simulink model "model"  (R2014a)
(part 5 of 5)

  T_166670638__/LConn2 -- _CN_166670638_220000_CN_166785368_220000/LConn2
  _CN_166670638_220000_CN_166785368_220000/LConn3 -- T_166670638__/LConn3 -- bus177/LConn1
  _CN_166670638_220000_CN_166785368_220000/RConn1 -- T_166785368__/LConn1 -- _CN_287217193_220000_CN_166785368_220000/LConn1
  _CN_166670638_220000_CN_166785368_220000/RConn2 -- T_166785368__/LConn2 -- _CN_287217193_220000_CN_166785368_220000/LConn2
  _CN_166670638_220000_CN_166785368_220000/RConn3 -- T_166785368__/LConn3 -- _CN_287217193_220000_CN_166785368_220000/LConn3 -- bus178/LConn1
  T_105834287__/LConn1 -- _CN_105834287_220000_CN_121056862_220000/RConn1
  T_105834287__/LConn2 -- _CN_105834287_220000_CN_121056862_220000/RConn2
  _CN_105834287_220000_CN_121056862_220000/RConn3 -- T_105834287__/LConn3 -- bus179/LConn1
  T_162167601__/LConn1 -- _CN_162167601_220000_CN_162167607_220000/LConn1
  T_162167601__/LConn2 -- _CN_162167601_220000_CN_162167607_220000/LConn2
  _CN_162167601_220000_CN_162167607_220000/LConn3 -- T_162167601__/LConn3 -- bus180/LConn1
  _CN_162167601_220000_CN_162167607_220000/RConn1 -- T_162167607__/LConn1 -- _CN_162167607_220000_CN_286930814_220000/LConn1 -- _CN_162167607_220000_CN_162378099_220000/RConn1
  _CN_162167601_220000_CN_162167607_220000/RConn2 -- T_162167607__/LConn2 -- _CN_162167607_220000_CN_286930814_220000/LConn2 -- _CN_162167607_220000_CN_162378099_220000/RConn2
  _CN_162167601_220000_CN_162167607_220000/RConn3 -- T_162167607__/LConn3 -- _CN_162167607_220000_CN_286930814_220000/LConn3 -- _CN_162167607_220000_CN_162378099_220000/RConn3 -- bus181/LConn1
  T_166785367__/LConn1 -- _CN_166670643_220000_CN_166785367_220000/RConn1
  T_166785367__/LConn2 -- _CN_166670643_220000_CN_166785367_220000/RConn2
  _CN_166670643_220000_CN_166785367_220000/RConn3 -- T_166785367__/LConn3 -- bus182/LConn1
  _CN_167981876_220000_CN_148003696_220000/LConn1 -- T_167981876_500000_/RConn1 -- L_167981876/LConn1
  _CN_167981876_220000_CN_148003696_220000/LConn2 -- T_167981876_500000_/RConn2 -- L_167981876/LConn2
  _CN_167981876_220000_CN_148003696_220000/LConn3 -- T_167981876_500000_/RConn3 -- L_167981876/LConn3 -- bus183/LConn1
  T_148003696__/LConn1 -- _CN_167981876_220000_CN_148003696_220000/RConn1
  T_148003696__/LConn2 -- _CN_167981876_220000_CN_148003696_220000/RConn2
  _CN_167981876_220000_CN_148003696_220000/RConn3 -- T_148003696__/LConn3 -- bus184/LConn1
  _CN_162167607_220000_CN_286930814_220000/RConn1 -- T_286930814__/LConn1 -- _CN_286930852_220000_CN_286930814_220000/RConn1
  _CN_162167607_220000_CN_286930814_220000/RConn2 -- T_286930814__/LConn2 -- _CN_286930852_220000_CN_286930814_220000/RConn2
  _CN_162167607_220000_CN_286930814_220000/RConn3 -- T_286930814__/LConn3 -- _CN_286930852_220000_CN_286930814_220000/RConn3 -- bus185/LConn1
  T_132430141__/LConn1 -- _CN_132430137_220000_CN_132430141_220000/RConn1
  T_132430141__/LConn2 -- _CN_132430137_220000_CN_132430141_220000/RConn2
  _CN_132430137_220000_CN_132430141_220000/RConn3 -- T_132430141__/LConn3 -- bus186/LConn1
  _CN_287217193_220000_CN_166670647_220000/LConn1 -- T_287217193__/LConn1 -- _CN_287217193_220000_CN_166785368_220000/RConn1 -- _CN_287217193_220000_CN_287217195_220000/LConn1
  _CN_287217193_220000_CN_166670647_220000/LConn2 -- T_287217193__/LConn2 -- _CN_287217193_220000_CN_166785368_220000/RConn2 -- _CN_287217193_220000_CN_287217195_220000/LConn2
  _CN_287217193_220000_CN_166670647_220000/LConn3 -- T_287217193__/LConn3 -- _CN_287217193_220000_CN_166785368_220000/RConn3 -- _CN_287217193_220000_CN_287217195_220000/LConn3 -- bus187/LConn1
  _CN_287217193_220000_CN_166670647_220000/RConn1 -- G_166670647_/RConn1 -- _CN_166670597_500000_CN_166670647_220000/LConn1
  _CN_287217193_220000_CN_166670647_220000/RConn2 -- G_166670647_/RConn2 -- _CN_166670597_500000_CN_166670647_220000/LConn2
  _CN_287217193_220000_CN_166670647_220000/RConn3 -- G_166670647_/RConn3 -- _CN_166670597_500000_CN_166670647_220000/LConn3 -- bus188/LConn1
  T_287217195__/LConn1 -- _CN_287217193_220000_CN_287217195_220000/RConn1
  T_287217195__/LConn2 -- _CN_287217193_220000_CN_287217195_220000/RConn2
  _CN_287217193_220000_CN_287217195_220000/RConn3 -- T_287217195__/LConn3 -- bus189/LConn1
  T_107081025_220000_/LConn1 -- _CN_107081025_220000_CN_107081068_220000/LConn1
  T_107081025_220000_/LConn2 -- _CN_107081025_220000_CN_107081068_220000/LConn2
  _CN_107081025_220000_CN_107081068_220000/LConn3 -- T_107081025_220000_/LConn3 -- bus190/LConn1
  _CN_107081025_220000_CN_107081068_220000/RConn1 -- G_107081068_吴泾热电站/RConn1 -- _CN_107081079_220000_CN_107081068_220000/LConn1
  _CN_107081025_220000_CN_107081068_220000/RConn2 -- G_107081068_吴泾热电站/RConn2 -- _CN_107081079_220000_CN_107081068_220000/LConn2
  _CN_107081025_220000_CN_107081068_220000/RConn3 -- G_107081068_吴泾热电站/RConn3 -- _CN_107081079_220000_CN_107081068_220000/LConn3 -- bus191/LConn1
  _CN_107025734_220000_CN_107025738_220000/LConn1 -- T_107025734__/LConn1 -- _CN_107025734_220000_CN_95805677_220000/RConn1
  _CN_107025734_220000_CN_107025738_220000/LConn2 -- T_107025734__/LConn2 -- _CN_107025734_220000_CN_95805677_220000/RConn2
  _CN_107025734_220000_CN_107025738_220000/LConn3 -- T_107025734__/LConn3 -- _CN_107025734_220000_CN_95805677_220000/RConn3 -- bus192/LConn1
  T_107025738__/LConn1 -- _CN_107025734_220000_CN_107025738_220000/RConn1
  T_107025738__/LConn2 -- _CN_107025734_220000_CN_107025738_220000/RConn2
  _CN_107025734_220000_CN_107025738_220000/RConn3 -- T_107025738__/LConn3 -- bus193/LConn1
  T_148630855__/LConn1 -- _CN_148630855_220000_CN_148630906_220000/LConn1
  T_148630855__/LConn2 -- _CN_148630855_220000_CN_148630906_220000/LConn2
  _CN_148630855_220000_CN_148630906_220000/LConn3 -- T_148630855__/LConn3 -- bus194/LConn1
  T_148630906__/LConn1 -- _CN_148630855_220000_CN_148630906_220000/RConn1
  T_148630906__/LConn2 -- _CN_148630855_220000_CN_148630906_220000/RConn2
  _CN_148630855_220000_CN_148630906_220000/RConn3 -- T_148630906__/LConn3 -- bus195/LConn1
  _CN_163357515_220000_CN_165791616_220000/LConn1 -- T_163357515__/RConn1 -- L_163357515/LConn1
  _CN_163357515_220000_CN_165791616_220000/LConn2 -- T_163357515__/RConn2 -- L_163357515/LConn2
  _CN_163357515_220000_CN_165791616_220000/LConn3 -- T_163357515__/RConn3 -- L_163357515/LConn3 -- bus196/LConn1
  T_165791616__/LConn1 -- _CN_163357515_220000_CN_165791616_220000/RConn1
  T_165791616__/LConn2 -- _CN_163357515_220000_CN_165791616_220000/RConn2
  _CN_163357515_220000_CN_165791616_220000/RConn3 -- T_165791616__/LConn3 -- bus197/LConn1
  _CN_355642647_220000_CN_313585533_220000/RConn1 -- T_313585533_220000_/LConn1 -- _CN_313585532_220000_CN_313585533_220000/RConn1
  _CN_355642647_220000_CN_313585533_220000/RConn2 -- T_313585533_220000_/LConn2 -- _CN_313585532_220000_CN_313585533_220000/RConn2
  _CN_355642647_220000_CN_313585533_220000/RConn3 -- T_313585533_220000_/LConn3 -- _CN_313585532_220000_CN_313585533_220000/RConn3 -- bus198/LConn1
  T_439464430__/LConn1 -- _CN_355642647_220000_CN_439464430_220000/RConn1
  T_439464430__/LConn2 -- _CN_355642647_220000_CN_439464430_220000/RConn2
  _CN_355642647_220000_CN_439464430_220000/RConn3 -- T_439464430__/LConn3 -- bus199/LConn1
  T_276589719__/LConn1 -- _CN_312789337_220000_CN_276589719_220000/RConn1
  T_276589719__/LConn2 -- _CN_312789337_220000_CN_276589719_220000/RConn2
  _CN_312789337_220000_CN_276589719_220000/RConn3 -- T_276589719__/LConn3 -- bus200/LConn1
  T_107025757_220000_/LConn1 -- _CN_107025757_220000_CN_95805677_220000/RConn1
  T_107025757_220000_/LConn2 -- _CN_107025757_220000_CN_95805677_220000/RConn2
  _CN_107025757_220000_CN_95805677_220000/RConn3 -- T_107025757_220000_/LConn3 -- bus201/LConn1
  T_137158504_220000_/LConn1 -- _CN_137158504_220000_CN_373557043_220000/LConn1
  T_137158504_220000_/LConn2 -- _CN_137158504_220000_CN_373557043_220000/LConn2
  _CN_137158504_220000_CN_373557043_220000/LConn3 -- T_137158504_220000_/LConn3 -- bus202/LConn1
  G_373557043_/RConn1 -- _CN_137158504_220000_CN_373557043_220000/RConn1
  G_373557043_/RConn2 -- _CN_137158504_220000_CN_373557043_220000/RConn2
  _CN_137158504_220000_CN_373557043_220000/RConn3 -- G_373557043_/RConn3 -- bus203/LConn1
  T_286930806__/LConn1 -- _CN_286930806_220000_CN_286930848_220000/LConn1
  T_286930806__/LConn2 -- _CN_286930806_220000_CN_286930848_220000/LConn2
  _CN_286930806_220000_CN_286930848_220000/LConn3 -- T_286930806__/LConn3 -- bus204/LConn1
  _CN_286930806_220000_CN_286930848_220000/RConn1 -- T_286930848__/LConn1 -- _CN_286930848_220000_CN_286930851_220000/LConn1
  _CN_286930806_220000_CN_286930848_220000/RConn2 -- T_286930848__/LConn2 -- _CN_286930848_220000_CN_286930851_220000/LConn2
  _CN_286930806_220000_CN_286930848_220000/RConn3 -- T_286930848__/LConn3 -- _CN_286930848_220000_CN_286930851_220000/LConn3 -- bus205/LConn1
  _CN_107081079_220000_CN_107081068_220000/RConn1 -- T_107081079_220000_/LConn1 -- _CN_107081079_220000_CN_95805677_220000/RConn1
  _CN_107081079_220000_CN_107081068_220000/RConn2 -- T_107081079_220000_/LConn2 -- _CN_107081079_220000_CN_95805677_220000/RConn2
  _CN_107081079_220000_CN_107081068_220000/RConn3 -- T_107081079_220000_/LConn3 -- _CN_107081079_220000_CN_95805677_220000/RConn3 -- bus206/LConn1
  T_201195907_220000_/LConn1 -- _CN_201195906_220000_CN_201195907_220000/RConn1
  T_201195907_220000_/LConn2 -- _CN_201195906_220000_CN_201195907_220000/RConn2
  _CN_201195906_220000_CN_201195907_220000/RConn3 -- T_201195907_220000_/LConn3 -- bus207/LConn1
  _CN_283658124_220000_CN_284090317_220000/LConn1 -- T_283658124__/RConn1 -- L_283658124/LConn1
  _CN_283658124_220000_CN_284090317_220000/LConn2 -- T_283658124__/RConn2 -- L_283658124/LConn2
  _CN_283658124_220000_CN_284090317_220000/LConn3 -- T_283658124__/RConn3 -- L_283658124/LConn3 -- bus208/LConn1
  _CN_283658124_220000_CN_284090317_220000/RConn1 -- T_284090317__/LConn1 -- _CN_284090317_220000_CN_284090323_220000/LConn1
  _CN_283658124_220000_CN_284090317_220000/RConn2 -- T_284090317__/LConn2 -- _CN_284090317_220000_CN_284090323_220000/LConn2
  _CN_283658124_220000_CN_284090317_220000/RConn3 -- T_284090317__/LConn3 -- _CN_284090317_220000_CN_284090323_220000/LConn3 -- bus209/LConn1
  _CN_128731545_220000_CN_132311997_220000/LConn1 -- T_128731545_220000_/LConn1 -- _CN_128731545_220000_CN_132312010_220000/RConn1 -- _CN_128731545_220000_CN_128731546_220000/RConn1
  _CN_128731545_220000_CN_132311997_220000/LConn2 -- T_128731545_220000_/LConn2 -- _CN_128731545_220000_CN_132312010_220000/RConn2 -- _CN_128731545_220000_CN_128731546_220000/RConn2
  _CN_128731545_220000_CN_132311997_220000/LConn3 -- T_128731545_220000_/LConn3 -- _CN_128731545_220000_CN_132312010_220000/RConn3 -- bus210/LConn1 -- _CN_128731545_220000_CN_128731546_220000/RConn3
  _CN_128731545_220000_CN_132311997_220000/RConn1 -- T_132311997_220000_/LConn1 -- _CN_132311997_220000_CN_132312010_220000/RConn1
  _CN_128731545_220000_CN_132311997_220000/RConn2 -- T_132311997_220000_/LConn2 -- _CN_132311997_220000_CN_132312010_220000/RConn2
  _CN_128731545_220000_CN_132311997_220000/RConn3 -- T_132311997_220000_/LConn3 -- _CN_132311997_220000_CN_132312010_220000/RConn3 -- bus211/LConn1
  T_286930851__/LConn1 -- _CN_286930848_220000_CN_286930851_220000/RConn1
  T_286930851__/LConn2 -- _CN_286930848_220000_CN_286930851_220000/RConn2
  _CN_286930848_220000_CN_286930851_220000/RConn3 -- T_286930851__/LConn3 -- bus212/LConn1
  T_223960988__/LConn1 -- _CN_223960988_220000_CN_337055172_220000/LConn1
  T_223960988__/LConn2 -- _CN_223960988_220000_CN_337055172_220000/LConn2
  _CN_223960988_220000_CN_337055172_220000/LConn3 -- T_223960988__/LConn3 -- bus213/LConn1
  T_337055172_500000_/LConn1 -- _CN_223960988_220000_CN_337055172_220000/RConn1
  T_337055172_500000_/LConn2 -- _CN_223960988_220000_CN_337055172_220000/RConn2
  _CN_223960988_220000_CN_337055172_220000/RConn3 -- T_337055172_500000_/LConn3 -- bus214/LConn1
  T_314318262_220000_/LConn1 -- _CN_314318262_220000_CN_314288467_220000/RConn1
  T_314318262_220000_/LConn2 -- _CN_314318262_220000_CN_314288467_220000/RConn2
  _CN_314318262_220000_CN_314288467_220000/RConn3 -- T_314318262_220000_/LConn3 -- bus215/LConn1
  T_284090323__/LConn1 -- _CN_284090317_220000_CN_284090323_220000/RConn1
  T_284090323__/LConn2 -- _CN_284090317_220000_CN_284090323_220000/RConn2
  _CN_284090317_220000_CN_284090323_220000/RConn3 -- T_284090323__/LConn3 -- bus216/LConn1
  T_163985922__/LConn1 -- _CN_163985922_500000_CN_127871762_500000/LConn1
  T_163985922__/LConn2 -- _CN_163985922_500000_CN_127871762_500000/LConn2
  _CN_163985922_500000_CN_127871762_500000/LConn3 -- T_163985922__/LConn3 -- bus217/LConn1
  T_127871762_500000_/LConn1 -- _CN_163985922_500000_CN_127871762_500000/RConn1
  T_127871762_500000_/LConn2 -- _CN_163985922_500000_CN_127871762_500000/RConn2
  _CN_163985922_500000_CN_127871762_500000/RConn3 -- T_127871762_500000_/LConn3 -- bus218/LConn1
  _CN_287200264_500000_CN_312588760_500000/LConn1 -- T_287200264__/LConn1 -- _CN_287200264_500000_CN_28939657_500000/LConn1 -- _CN_287200264_500000_CN_287132220_500000/LConn1
  _CN_287200264_500000_CN_312588760_500000/LConn2 -- T_287200264__/LConn2 -- _CN_287200264_500000_CN_28939657_500000/LConn2 -- _CN_287200264_500000_CN_287132220_500000/LConn2
  _CN_287200264_500000_CN_312588760_500000/LConn3 -- T_287200264__/LConn3 -- _CN_287200264_500000_CN_28939657_500000/LConn3 -- _CN_287200264_500000_CN_287132220_500000/LConn3 -- bus219/LConn1
  T_312588760_500000_/LConn1 -- _CN_287200264_500000_CN_312588760_500000/RConn1
  T_312588760_500000_/LConn2 -- _CN_287200264_500000_CN_312588760_500000/RConn2
  _CN_287200264_500000_CN_312588760_500000/RConn3 -- T_312588760_500000_/LConn3 -- bus220/LConn1
  _CN_287200264_500000_CN_28939657_500000/RConn1 -- G_28939657_田湾核电站/RConn1 -- _CN_287088780_500000_CN_28939657_500000/LConn1
  _CN_287200264_500000_CN_28939657_500000/RConn2 -- G_28939657_田湾核电站/RConn2 -- _CN_287088780_500000_CN_28939657_500000/LConn2
  _CN_287200264_500000_CN_28939657_500000/RConn3 -- G_28939657_田湾核电站/RConn3 -- _CN_287088780_500000_CN_28939657_500000/LConn3 -- bus221/LConn1
  _CN_287200264_500000_CN_287132220_500000/RConn1 -- T_287132220__/LConn1 -- _CN_287132220_500000_CN_287088780_500000/LConn1
  _CN_287200264_500000_CN_287132220_500000/RConn2 -- T_287132220__/LConn2 -- _CN_287132220_500000_CN_287088780_500000/LConn2
  _CN_287200264_500000_CN_287132220_500000/RConn3 -- T_287132220__/LConn3 -- _CN_287132220_500000_CN_287088780_500000/LConn3 -- bus222/LConn1
  T_194636809__/LConn1 -- _CN_194636809_500000_CN_192701020_500000/LConn1
  T_194636809__/LConn2 -- _CN_194636809_500000_CN_192701020_500000/LConn2
  _CN_194636809_500000_CN_192701020_500000/LConn3 -- T_194636809__/LConn3 -- bus223/LConn1
  T_192701020_500000_/LConn1 -- _CN_194636809_500000_CN_192701020_500000/RConn1
  T_192701020_500000_/LConn2 -- _CN_194636809_500000_CN_192701020_500000/RConn2
  _CN_194636809_500000_CN_192701020_500000/RConn3 -- T_192701020_500000_/LConn3 -- bus224/LConn1
  T_328518154_500000_/LConn1 -- _CN_328518154_500000_CN_275985691_500000/LConn1
  T_328518154_500000_/LConn2 -- _CN_328518154_500000_CN_275985691_500000/LConn2
  _CN_328518154_500000_CN_275985691_500000/LConn3 -- T_328518154_500000_/LConn3 -- bus225/LConn1
  _CN_328518154_500000_CN_275985691_500000/RConn1 -- T_275985691_500000_房山变电站/LConn1 -- 昌平一房山500kV紧_CN_275985691_500000_CN_276719460_500000/LConn1
  _CN_328518154_500000_CN_275985691_500000/RConn2 -- T_275985691_500000_房山变电站/LConn2 -- 昌平一房山500kV紧_CN_275985691_500000_CN_276719460_500000/LConn2
  _CN_328518154_500000_CN_275985691_500000/RConn3 -- T_275985691_500000_房山变电站/LConn3 -- 昌平一房山500kV紧_CN_275985691_500000_CN_276719460_500000/LConn3 -- bus226/LConn1
  T_315071500_500000_/LConn1 -- _CN_315071500_500000_CN_147855286_500000/LConn1
  T_315071500_500000_/LConn2 -- _CN_315071500_500000_CN_147855286_500000/LConn2
  _CN_315071500_500000_CN_147855286_500000/LConn3 -- T_315071500_500000_/LConn3 -- bus227/LConn1
  G_147855286_/RConn1 -- _CN_315071500_500000_CN_147855286_500000/RConn1
  G_147855286_/RConn2 -- _CN_315071500_500000_CN_147855286_500000/RConn2
  _CN_315071500_500000_CN_147855286_500000/RConn3 -- G_147855286_/RConn3 -- bus228/LConn1
  _CN_349963792_500000_CN_143214751_500000/LConn1 -- T_349963792__/LConn1 -- _CN_349963792_500000_CN_281631619_500000/LConn1 -- _CN_349963792_500000_CN_281631607_500000/LConn1
  _CN_349963792_500000_CN_143214751_500000/LConn2 -- T_349963792__/LConn2 -- _CN_349963792_500000_CN_281631619_500000/LConn2 -- _CN_349963792_500000_CN_281631607_500000/LConn2
  _CN_349963792_500000_CN_143214751_500000/LConn3 -- T_349963792__/LConn3 -- _CN_349963792_500000_CN_281631619_500000/LConn3 -- _CN_349963792_500000_CN_281631607_500000/LConn3 -- bus229/LConn1
  _CN_349963792_500000_CN_143214751_500000/RConn1 -- T_143214751__/LConn1 -- _CN_143214751_500000_CN_181221620_500000/LConn1
  _CN_349963792_500000_CN_143214751_500000/RConn2 -- T_143214751__/LConn2 -- _CN_143214751_500000_CN_181221620_500000/LConn2
  _CN_349963792_500000_CN_143214751_500000/RConn3 -- T_143214751__/LConn3 -- _CN_143214751_500000_CN_181221620_500000/LConn3 -- bus230/LConn1
  T_281631619__/LConn1 -- _CN_349963792_500000_CN_281631619_500000/RConn1
  T_281631619__/LConn2 -- _CN_349963792_500000_CN_281631619_500000/RConn2
  _CN_349963792_500000_CN_281631619_500000/RConn3 -- T_281631619__/LConn3 -- bus231/LConn1
  _CN_349963792_500000_CN_281631607_500000/RConn1 -- T_281631607__/LConn1 -- _CN_281631607_500000_CN_163357534_500000/LConn1
  _CN_349963792_500000_CN_281631607_500000/RConn2 -- T_281631607__/LConn2 -- _CN_281631607_500000_CN_163357534_500000/LConn2
  _CN_349963792_500000_CN_281631607_500000/RConn3 -- T_281631607__/LConn3 -- _CN_281631607_500000_CN_163357534_500000/LConn3 -- bus232/LConn1
  T_161803803_500000_/LConn1 -- _CN_161803803_500000_CN_259721828_500000/LConn1
  T_161803803_500000_/LConn2 -- _CN_161803803_500000_CN_259721828_500000/LConn2
  _CN_161803803_500000_CN_259721828_500000/LConn3 -- T_161803803_500000_/LConn3 -- bus233/LConn1
  _CN_161803803_500000_CN_259721828_500000/RConn1 -- T_259721828_500000_/LConn1 -- _CN_259721828_500000_CN_325720933_500000/LConn1 -- _CN_259721828_500000_CN_314883039_500000/LConn1 -- _CN_259721828_500000_CN_314866321_500000/LConn1 -- _CN_319236194_500000_CN_259721828_500000/LConn1
  _CN_161803803_500000_CN_259721828_500000/RConn2 -- T_259721828_500000_/LConn2 -- _CN_259721828_500000_CN_325720933_500000/LConn2 -- _CN_259721828_500000_CN_314883039_500000/LConn2 -- _CN_259721828_500000_CN_314866321_500000/LConn2 -- _CN_319236194_500000_CN_259721828_500000/LConn2
  _CN_161803803_500000_CN_259721828_500000/RConn3 -- T_259721828_500000_/LConn3 -- _CN_259721828_500000_CN_325720933_500000/LConn3 -- _CN_259721828_500000_CN_314883039_500000/LConn3 -- _CN_259721828_500000_CN_314866321_500000/LConn3 -- bus234/LConn1 -- _CN_319236194_500000_CN_259721828_500000/LConn3
  T_328430431_500000_/LConn1 -- _CN_328430431_500000_CN_212792929_500000/LConn1
  T_328430431_500000_/LConn2 -- _CN_328430431_500000_CN_212792929_500000/LConn2
  _CN_328430431_500000_CN_212792929_500000/LConn3 -- T_328430431_500000_/LConn3 -- bus235/LConn1
  _CN_328430431_500000_CN_212792929_500000/RConn1 -- T_212792929__/LConn1 -- _CN_212792929_500000_CN_302492014_500000/LConn1
  _CN_328430431_500000_CN_212792929_500000/RConn2 -- T_212792929__/LConn2 -- _CN_212792929_500000_CN_302492014_500000/LConn2
  _CN_328430431_500000_CN_212792929_500000/RConn3 -- T_212792929__/LConn3 -- _CN_212792929_500000_CN_302492014_500000/LConn3 -- bus236/LConn1
  _CN_287132220_500000_CN_287088780_500000/RConn1 -- T_287088780_500000_/LConn1 -- _CN_287088780_500000_CN_28939657_500000/RConn1 -- _CN_287088780_500000_CN_287076644_500000/LConn1 -- _CN_287088780_500000_CN_287076645_500000/LConn1
  _CN_287132220_500000_CN_287088780_500000/RConn2 -- T_287088780_500000_/LConn2 -- _CN_287088780_500000_CN_28939657_500000/RConn2 -- _CN_287088780_500000_CN_287076644_500000/LConn2 -- _CN_287088780_500000_CN_287076645_500000/LConn2
  _CN_287132220_500000_CN_287088780_500000/RConn3 -- T_287088780_500000_/LConn3 -- _CN_287088780_500000_CN_28939657_500000/RConn3 -- _CN_287088780_500000_CN_287076644_500000/LConn3 -- _CN_287088780_500000_CN_287076645_500000/LConn3 -- bus237/LConn1
  T_275706430_500000_昌平变电站/LConn1 -- _CN_275706430_500000_CN_148727570_500000/LConn1
  T_275706430_500000_昌平变电站/LConn2 -- _CN_275706430_500000_CN_148727570_500000/LConn2
  _CN_275706430_500000_CN_148727570_500000/LConn3 -- T_275706430_500000_昌平变电站/LConn3 -- bus238/LConn1
  _CN_275706430_500000_CN_148727570_500000/RConn1 -- T_148727570_500000_/LConn1 -- _CN_148727570_500000_CN_278062437_500000/LConn1 -- _CN_148727570_500000_CN_312852542_500000/LConn1
  _CN_275706430_500000_CN_148727570_500000/RConn2 -- T_148727570_500000_/LConn2 -- _CN_148727570_500000_CN_278062437_500000/LConn2 -- _CN_148727570_500000_CN_312852542_500000/LConn2
  _CN_275706430_500000_CN_148727570_500000/RConn3 -- T_148727570_500000_/LConn3 -- _CN_148727570_500000_CN_278062437_500000/LConn3 -- _CN_148727570_500000_CN_312852542_500000/LConn3 -- bus239/LConn1
  _CN_317023804_500000_CN_147744835_500000/LConn1 -- T_317023804_500000_/LConn1 -- _CN_317023804_500000_CN_251393861_500000/LConn1
  _CN_317023804_500000_CN_147744835_500000/LConn2 -- T_317023804_500000_/LConn2 -- _CN_317023804_500000_CN_251393861_500000/LConn2
  _CN_317023804_500000_CN_147744835_500000/LConn3 -- T_317023804_500000_/LConn3 -- _CN_317023804_500000_CN_251393861_500000/LConn3 -- bus240/LConn1
  _CN_317023804_500000_CN_147744835_500000/RConn1 -- T_147744835_500000_/LConn1 -- _CN_147744835_500000_CN_188829044_500000/LConn1
  _CN_317023804_500000_CN_147744835_500000/RConn2 -- T_147744835_500000_/LConn2 -- _CN_147744835_500000_CN_188829044_500000/LConn2
  _CN_317023804_500000_CN_147744835_500000/RConn3 -- T_147744835_500000_/LConn3 -- _CN_147744835_500000_CN_188829044_500000/LConn3 -- bus241/LConn1
  _CN_317023804_500000_CN_251393861_500000/RConn1 -- T_251393861_500000_/LConn1 -- _CN_251393861_500000_CN_251522340_500000/LConn1
  _CN_317023804_500000_CN_251393861_500000/RConn2 -- T_251393861_500000_/LConn2 -- _CN_251393861_500000_CN_251522340_500000/LConn2
  _CN_317023804_500000_CN_251393861_500000/RConn3 -- T_251393861_500000_/LConn3 -- _CN_251393861_500000_CN_251522340_500000/LConn3 -- bus242/LConn1
  _CN_147744835_500000_CN_188829044_500000/RConn1 -- T_188829044_500000_/LConn1 -- _CN_188829044_500000_CN_147708063_500000/LConn1
  _CN_147744835_500000_CN_188829044_500000/RConn2 -- T_188829044_500000_/LConn2 -- _CN_188829044_500000_CN_147708063_500000/LConn2
  _CN_147744835_500000_CN_188829044_500000/RConn3 -- T_188829044_500000_/LConn3 -- _CN_188829044_500000_CN_147708063_500000/LConn3 -- bus243/LConn1
  _CN_313528393_500000_CN_313528394_500000/LConn1 -- T_313528393_500000_/LConn1 -- _CN_313528393_500000_CN_304003393_500000/LConn1 -- _CN_313528393_500000_CN_313528427_500000/LConn1
  _CN_313528393_500000_CN_313528394_500000/LConn2 -- T_313528393_500000_/LConn2 -- _CN_313528393_500000_CN_304003393_500000/LConn2 -- _CN_313528393_500000_CN_313528427_500000/LConn2
  _CN_313528393_500000_CN_313528394_500000/LConn3 -- T_313528393_500000_/LConn3 -- _CN_313528393_500000_CN_304003393_500000/LConn3 -- _CN_313528393_500000_CN_313528427_500000/LConn3 -- bus244/LConn1
  T_313528394_500000_/LConn1 -- _CN_313528393_500000_CN_313528394_500000/RConn1
  T_313528394_500000_/LConn2 -- _CN_313528393_500000_CN_313528394_500000/RConn2
  _CN_313528393_500000_CN_313528394_500000/RConn3 -- T_313528394_500000_/LConn3 -- bus245/LConn1
  T_304003393_500000_/LConn1 -- _CN_313528393_500000_CN_304003393_500000/RConn1
  T_304003393_500000_/LConn2 -- _CN_313528393_500000_CN_304003393_500000/RConn2
  _CN_313528393_500000_CN_304003393_500000/RConn3 -- T_304003393_500000_/LConn3 -- bus246/LConn1
  _CN_313528393_500000_CN_313528427_500000/RConn1 -- T_313528427_500000_/LConn1 -- _CN_313528427_500000_CN_261427501_500000/LConn1
  _CN_313528393_500000_CN_313528427_500000/RConn2 -- T_313528427_500000_/LConn2 -- _CN_313528427_500000_CN_261427501_500000/LConn2
  _CN_313528393_500000_CN_313528427_500000/RConn3 -- T_313528427_500000_/LConn3 -- _CN_313528427_500000_CN_261427501_500000/LConn3 -- bus247/LConn1
  _CN_319236194_500000_CN_259721828_500000/RConn1 -- T_319236194_500000_/LConn1 -- _CN_319236194_500000_CN_321597229_500000/LConn1
  _CN_319236194_500000_CN_259721828_500000/RConn2 -- T_319236194_500000_/LConn2 -- _CN_319236194_500000_CN_321597229_500000/LConn2
  _CN_319236194_500000_CN_259721828_500000/RConn3 -- T_319236194_500000_/LConn3 -- _CN_319236194_500000_CN_321597229_500000/LConn3 -- bus248/LConn1
  _CN_319236194_500000_CN_321597229_500000/RConn1 -- T_321597229_500000_/LConn1 -- _CN_321597229_500000_CN_302492014_500000/LConn1
  _CN_319236194_500000_CN_321597229_500000/RConn2 -- T_321597229_500000_/LConn2 -- _CN_321597229_500000_CN_302492014_500000/LConn2
  _CN_319236194_500000_CN_321597229_500000/RConn3 -- T_321597229_500000_/LConn3 -- _CN_321597229_500000_CN_302492014_500000/LConn3 -- bus249/LConn1
  _CN_264811102_500000_CN_201195906_500000/LConn1 -- T_264811102_500000_/LConn1 -- _CN_264811102_500000_CN_221891107_500000/LConn1
  _CN_264811102_500000_CN_201195906_500000/LConn2 -- T_264811102_500000_/LConn2 -- _CN_264811102_500000_CN_221891107_500000/LConn2
  _CN_264811102_500000_CN_201195906_500000/LConn3 -- T_264811102_500000_/LConn3 -- _CN_264811102_500000_CN_221891107_500000/LConn3 -- bus250/LConn1
  T_201195906_500000_/LConn1 -- _CN_264811102_500000_CN_201195906_500000/RConn1
  T_201195906_500000_/LConn2 -- _CN_264811102_500000_CN_201195906_500000/RConn2
  _CN_264811102_500000_CN_201195906_500000/RConn3 -- T_201195906_500000_/LConn3 -- bus251/LConn1
  _CN_264811102_500000_CN_221891107_500000/RConn1 -- G_221891107_/RConn1 -- _CN_135466215_500000_CN_221891107_500000/LConn1 -- _CN_277499262_500000_CN_221891107_500000/LConn1
  _CN_264811102_500000_CN_221891107_500000/RConn2 -- G_221891107_/RConn2 -- _CN_135466215_500000_CN_221891107_500000/LConn2 -- _CN_277499262_500000_CN_221891107_500000/LConn2
  _CN_264811102_500000_CN_221891107_500000/RConn3 -- G_221891107_/RConn3 -- _CN_135466215_500000_CN_221891107_500000/LConn3 -- _CN_277499262_500000_CN_221891107_500000/LConn3 -- bus252/LConn1
  _CN_212792929_500000_CN_302492014_500000/RConn1 -- T_302492014__/LConn1 -- _CN_321597229_500000_CN_302492014_500000/RConn1
  _CN_212792929_500000_CN_302492014_500000/RConn2 -- T_302492014__/LConn2 -- _CN_321597229_500000_CN_302492014_500000/RConn2
  _CN_212792929_500000_CN_302492014_500000/RConn3 -- T_302492014__/LConn3 -- _CN_321597229_500000_CN_302492014_500000/RConn3 -- bus253/LConn1
  _CN_128686690_500000_CN_151766812_500000/LConn1 -- T_128686690_500000_/LConn1 -- _CN_128686690_500000_CN_171491177_500000/LConn1 -- _CN_128686690_500000_CN_424682264_500000/LConn1 -- _CN_128686690_500000_CN_171491189_500000/LConn1
  _CN_128686690_500000_CN_151766812_500000/LConn2 -- T_128686690_500000_/LConn2 -- _CN_128686690_500000_CN_171491177_500000/LConn2 -- _CN_128686690_500000_CN_424682264_500000/LConn2 -- _CN_128686690_500000_CN_171491189_500000/LConn2
  _CN_128686690_500000_CN_151766812_500000/LConn3 -- T_128686690_500000_/LConn3 -- _CN_128686690_500000_CN_171491177_500000/LConn3 -- _CN_128686690_500000_CN_424682264_500000/LConn3 -- _CN_128686690_500000_CN_171491189_500000/LConn3 -- bus254/LConn1
  _CN_128686690_500000_CN_151766812_500000/RConn1 -- T_151766812_500000;220000_/LConn1 -- _CN_151766812_500000_CN_424682272_500000/LConn1
  _CN_128686690_500000_CN_151766812_500000/RConn2 -- T_151766812_500000;220000_/LConn2 -- _CN_151766812_500000_CN_424682272_500000/LConn2
  _CN_128686690_500000_CN_151766812_500000/RConn3 -- T_151766812_500000;220000_/LConn3 -- _CN_151766812_500000_CN_424682272_500000/LConn3 -- bus255/LConn1
  _CN_128686690_500000_CN_171491177_500000/RConn1 -- T_171491177_500000_漕泾/LConn1 -- _CN_132424981_500000_CN_171491177_500000/LConn1 -- _CN_171491177_500000_CN_171491178_500000/LConn1
  _CN_128686690_500000_CN_171491177_500000/RConn2 -- T_171491177_500000_漕泾/LConn2 -- _CN_132424981_500000_CN_171491177_500000/LConn2 -- _CN_171491177_500000_CN_171491178_500000/LConn2
  _CN_128686690_500000_CN_171491177_500000/RConn3 -- T_171491177_500000_漕泾/LConn3 -- _CN_132424981_500000_CN_171491177_500000/LConn3 -- _CN_171491177_500000_CN_171491178_500000/LConn3 -- bus256/LConn1
  T_424682264__/LConn1 -- _CN_128686690_500000_CN_424682264_500000/RConn1
  T_424682264__/LConn2 -- _CN_128686690_500000_CN_424682264_500000/RConn2
  _CN_128686690_500000_CN_424682264_500000/RConn3 -- T_424682264__/LConn3 -- bus257/LConn1
  T_171491189__/LConn1 -- _CN_128686690_500000_CN_171491189_500000/RConn1
  T_171491189__/LConn2 -- _CN_128686690_500000_CN_171491189_500000/RConn2
  _CN_128686690_500000_CN_171491189_500000/RConn3 -- T_171491189__/LConn3 -- bus258/LConn1
  T_313316283_500000_/LConn1 -- _CN_313316283_500000_CN_148104555_500000/LConn1
  T_313316283_500000_/LConn2 -- _CN_313316283_500000_CN_148104555_500000/LConn2
  _CN_313316283_500000_CN_148104555_500000/LConn3 -- T_313316283_500000_/LConn3 -- bus259/LConn1
  T_148104555__/LConn1 -- _CN_313316283_500000_CN_148104555_500000/RConn1
  T_148104555__/LConn2 -- _CN_313316283_500000_CN_148104555_500000/RConn2
  _CN_313316283_500000_CN_148104555_500000/RConn3 -- T_148104555__/LConn3 -- bus260/LConn1
  T_325720933_500000_/LConn1 -- _CN_259721828_500000_CN_325720933_500000/RConn1
  T_325720933_500000_/LConn2 -- _CN_259721828_500000_CN_325720933_500000/RConn2
  _CN_259721828_500000_CN_325720933_500000/RConn3 -- T_325720933_500000_/LConn3 -- bus261/LConn1
  _CN_259721828_500000_CN_314883039_500000/RConn1 -- T_314883039_500000_/LConn1 -- _CN_325720937_500000_CN_314883039_500000/LConn1
  _CN_259721828_500000_CN_314883039_500000/RConn2 -- T_314883039_500000_/LConn2 -- _CN_325720937_500000_CN_314883039_500000/LConn2
  _CN_259721828_500000_CN_314883039_500000/RConn3 -- T_314883039_500000_/LConn3 -- _CN_325720937_500000_CN_314883039_500000/LConn3 -- bus262/LConn1
  _CN_259721828_500000_CN_314866321_500000/RConn1 -- T_314866321_500000_/LConn1 -- _CN_325720937_500000_CN_314866321_500000/LConn1
  _CN_259721828_500000_CN_314866321_500000/RConn2 -- T_314866321_500000_/LConn2 -- _CN_325720937_500000_CN_314866321_500000/LConn2
  _CN_259721828_500000_CN_314866321_500000/RConn3 -- T_314866321_500000_/LConn3 -- _CN_325720937_500000_CN_314866321_500000/LConn3 -- bus263/LConn1
  T_317280360__/LConn1 -- _CN_317280360_500000_CN_327333768_500000/LConn1
  T_317280360__/LConn2 -- _CN_317280360_500000_CN_327333768_500000/LConn2
  _CN_317280360_500000_CN_327333768_500000/LConn3 -- T_317280360__/LConn3 -- bus264/LConn1
  _CN_317280360_500000_CN_327333768_500000/RConn1 -- T_327333768_500000_/LConn1 -- _CN_327333768_500000_CN_181090227_500000/LConn1
  _CN_317280360_500000_CN_327333768_500000/RConn2 -- T_327333768_500000_/LConn2 -- _CN_327333768_500000_CN_181090227_500000/LConn2
  _CN_317280360_500000_CN_327333768_500000/RConn3 -- T_327333768_500000_/LConn3 -- _CN_327333768_500000_CN_181090227_500000/LConn3 -- bus265/LConn1
  T_261427501__/LConn1 -- _CN_313528427_500000_CN_261427501_500000/RConn1
  T_261427501__/LConn2 -- _CN_313528427_500000_CN_261427501_500000/RConn2
  _CN_313528427_500000_CN_261427501_500000/RConn3 -- T_261427501__/LConn3 -- bus266/LConn1
  _CN_148727570_500000_CN_278062437_500000/RConn1 -- T_278062437__/LConn1 -- _CN_278062437_500000_CN_312852542_500000/LConn1
  _CN_148727570_500000_CN_278062437_500000/RConn2 -- T_278062437__/LConn2 -- _CN_278062437_500000_CN_312852542_500000/LConn2
  _CN_148727570_500000_CN_278062437_500000/RConn3 -- T_278062437__/LConn3 -- _CN_278062437_500000_CN_312852542_500000/LConn3 -- bus267/LConn1
  _CN_148727570_500000_CN_312852542_500000/RConn1 -- T_312852542_500000_/LConn1 -- _CN_135466215_500000_CN_312852542_500000/LConn1 -- _CN_278062437_500000_CN_312852542_500000/RConn1 -- _CN_277499262_500000_CN_312852542_500000/LConn1
  _CN_148727570_500000_CN_312852542_500000/RConn2 -- T_312852542_500000_/LConn2 -- _CN_135466215_500000_CN_312852542_500000/LConn2 -- _CN_278062437_500000_CN_312852542_500000/RConn2 -- _CN_277499262_500000_CN_312852542_500000/LConn2
  _CN_148727570_500000_CN_312852542_500000/RConn3 -- T_312852542_500000_/LConn3 -- _CN_135466215_500000_CN_312852542_500000/LConn3 -- _CN_278062437_500000_CN_312852542_500000/RConn3 -- _CN_277499262_500000_CN_312852542_500000/LConn3 -- bus268/LConn1
  _CN_325720937_500000_CN_314883039_500000/RConn1 -- T_325720937_500000_/LConn1 -- _CN_325720937_500000_CN_146077915_500000/LConn1 -- _CN_325720937_500000_CN_312922833_500000/LConn1 -- _CN_325720937_500000_CN_314866321_500000/RConn1
  _CN_325720937_500000_CN_314883039_500000/RConn2 -- T_325720937_500000_/LConn2 -- _CN_325720937_500000_CN_146077915_500000/LConn2 -- _CN_325720937_500000_CN_312922833_500000/LConn2 -- _CN_325720937_500000_CN_314866321_500000/RConn2
  _CN_325720937_500000_CN_314883039_500000/RConn3 -- T_325720937_500000_/LConn3 -- _CN_325720937_500000_CN_146077915_500000/LConn3 -- _CN_325720937_500000_CN_312922833_500000/LConn3 -- _CN_325720937_500000_CN_314866321_500000/RConn3 -- bus269/LConn1
  _CN_325720937_500000_CN_146077915_500000/RConn1 -- T_146077915__/LConn1 -- _CN_312922832_500000_CN_146077915_500000/LConn1 -- _CN_146077915_500000_CN_133523400_500000/LConn1
  _CN_325720937_500000_CN_146077915_500000/RConn2 -- T_146077915__/LConn2 -- _CN_312922832_500000_CN_146077915_500000/LConn2 -- _CN_146077915_500000_CN_133523400_500000/LConn2
  _CN_325720937_500000_CN_146077915_500000/RConn3 -- T_146077915__/LConn3 -- _CN_312922832_500000_CN_146077915_500000/LConn3 -- _CN_146077915_500000_CN_133523400_500000/LConn3 -- bus270/LConn1
  T_312922833_500000_/LConn1 -- _CN_325720937_500000_CN_312922833_500000/RConn1
  T_312922833_500000_/LConn2 -- _CN_325720937_500000_CN_312922833_500000/RConn2
  _CN_325720937_500000_CN_312922833_500000/RConn3 -- T_312922833_500000_/LConn3 -- bus271/LConn1
  _CN_132424981_500000_CN_132443907_500000/LConn1 -- T_132424981__/LConn1 -- _CN_132424981_500000_CN_171491177_500000/RConn1 -- _CN_132424981_500000_CN_132424995_500000/LConn1
  _CN_132424981_500000_CN_132443907_500000/LConn2 -- T_132424981__/LConn2 -- _CN_132424981_500000_CN_171491177_500000/RConn2 -- _CN_132424981_500000_CN_132424995_500000/LConn2
  _CN_132424981_500000_CN_132443907_500000/LConn3 -- T_132424981__/LConn3 -- _CN_132424981_500000_CN_171491177_500000/RConn3 -- bus272/LConn1 -- _CN_132424981_500000_CN_132424995_500000/LConn3
  T_132443907__/LConn1 -- _CN_132424981_500000_CN_132443907_500000/RConn1
  T_132443907__/LConn2 -- _CN_132424981_500000_CN_132443907_500000/RConn2
  _CN_132424981_500000_CN_132443907_500000/RConn3 -- T_132443907__/LConn3 -- bus273/LConn1
  T_132424995__/LConn1 -- _CN_132424981_500000_CN_132424995_500000/RConn1
  T_132424995__/LConn2 -- _CN_132424981_500000_CN_132424995_500000/RConn2
  _CN_132424981_500000_CN_132424995_500000/RConn3 -- T_132424995__/LConn3 -- bus274/LConn1
  _CN_323106411_500000_CN_322456943_500000/LConn1 -- T_323106411_220000_/LConn1 -- _CN_323106411_500000_CN_299934546_500000/LConn1 -- _CN_323106411_500000_CN_323032993_500000/LConn1 -- _CN_323106411_500000_CN_322892827_500000/LConn1 -- _CN_323106411_500000_CN_323016571_500000/LConn1
  _CN_323106411_500000_CN_322456943_500000/LConn2 -- T_323106411_220000_/LConn2 -- _CN_323106411_500000_CN_299934546_500000/LConn2 -- _CN_323106411_500000_CN_323032993_500000/LConn2 -- _CN_323106411_500000_CN_322892827_500000/LConn2 -- _CN_323106411_500000_CN_323016571_500000/LConn2
  _CN_323106411_500000_CN_322456943_500000/LConn3 -- T_323106411_220000_/LConn3 -- _CN_323106411_500000_CN_299934546_500000/LConn3 -- _CN_323106411_500000_CN_323032993_500000/LConn3 -- _CN_323106411_500000_CN_322892827_500000/LConn3 -- _CN_323106411_500000_CN_323016571_500000/LConn3 -- bus275/LConn1
  G_322456943_嘉兴发电厂/RConn1 -- _CN_323106411_500000_CN_322456943_500000/RConn1
  G_322456943_嘉兴发电厂/RConn2 -- _CN_323106411_500000_CN_322456943_500000/RConn2
  _CN_323106411_500000_CN_322456943_500000/RConn3 -- G_322456943_嘉兴发电厂/RConn3 -- bus276/LConn1
  G_299934546_方家山核电站/RConn1 -- _CN_323106411_500000_CN_299934546_500000/RConn1
  G_299934546_方家山核电站/RConn2 -- _CN_323106411_500000_CN_299934546_500000/RConn2
  _CN_323106411_500000_CN_299934546_500000/RConn3 -- G_299934546_方家山核电站/RConn3 -- bus277/LConn1
  T_323032993_500000_/LConn1 -- _CN_323106411_500000_CN_323032993_500000/RConn1
  T_323032993_500000_/LConn2 -- _CN_323106411_500000_CN_323032993_500000/RConn2
  _CN_323106411_500000_CN_323032993_500000/RConn3 -- T_323032993_500000_/LConn3 -- bus278/LConn1
  T_322892827_500000_/LConn1 -- _CN_323106411_500000_CN_322892827_500000/RConn1
  T_322892827_500000_/LConn2 -- _CN_323106411_500000_CN_322892827_500000/RConn2
  _CN_323106411_500000_CN_322892827_500000/RConn3 -- T_322892827_500000_/LConn3 -- bus279/LConn1
  _CN_323106411_500000_CN_323016571_500000/RConn1 -- T_323016571_500000_/LConn1 -- _CN_232408714_500000_CN_323016571_500000/LConn1 -- _CN_424682265_500000_CN_323016571_500000/LConn1
  _CN_323106411_500000_CN_323016571_500000/RConn2 -- T_323016571_500000_/LConn2 -- _CN_232408714_500000_CN_323016571_500000/LConn2 -- _CN_424682265_500000_CN_323016571_500000/LConn2
  _CN_323106411_500000_CN_323016571_500000/RConn3 -- T_323016571_500000_/LConn3 -- _CN_232408714_500000_CN_323016571_500000/LConn3 -- _CN_424682265_500000_CN_323016571_500000/LConn3 -- bus280/LConn1
  _CN_136348806_500000_CN_133523400_500000/LConn1 -- T_136348806_500000_/LConn1 -- _CN_136348806_500000_CN_279809227_500000/LConn1
  _CN_136348806_500000_CN_133523400_500000/LConn2 -- T_136348806_500000_/LConn2 -- _CN_136348806_500000_CN_279809227_500000/LConn2
  _CN_136348806_500000_CN_133523400_500000/LConn3 -- T_136348806_500000_/LConn3 -- _CN_136348806_500000_CN_279809227_500000/LConn3 -- bus281/LConn1
  _CN_136348806_500000_CN_133523400_500000/RConn1 -- T_133523400_500000_/LConn1 -- _CN_146077915_500000_CN_133523400_500000/RConn1
  _CN_136348806_500000_CN_133523400_500000/RConn2 -- T_133523400_500000_/LConn2 -- _CN_146077915_500000_CN_133523400_500000/RConn2
  _CN_136348806_500000_CN_133523400_500000/RConn3 -- T_133523400_500000_/LConn3 -- _CN_146077915_500000_CN_133523400_500000/RConn3 -- bus282/LConn1
  T_279809227__/LConn1 -- _CN_136348806_500000_CN_279809227_500000/RConn1
  T_279809227__/LConn2 -- _CN_136348806_500000_CN_279809227_500000/RConn2
  _CN_136348806_500000_CN_279809227_500000/RConn3 -- T_279809227__/LConn3 -- bus283/LConn1
  _CN_232408714_500000_CN_323698983_500000/LConn1 -- T_232408714_500000_里木栅500KV超高压变电站/LConn1 -- _CN_232408714_500000_CN_323965697_500000/LConn1 -- _CN_232408714_500000_CN_323880677_500000/LConn1 -- _CN_232408714_500000_CN_323016571_500000/RConn1
  _CN_232408714_500000_CN_323698983_500000/LConn2 -- T_232408714_500000_里木栅500KV超高压变电站/LConn2 -- _CN_232408714_500000_CN_323965697_500000/LConn2 -- _CN_232408714_500000_CN_323880677_500000/LConn2 -- _CN_232408714_500000_CN_323016571_500000/RConn2
  _CN_232408714_500000_CN_323698983_500000/LConn3 -- T_232408714_500000_里木栅500KV超高压变电站/LConn3 -- _CN_232408714_500000_CN_323965697_500000/LConn3 -- _CN_232408714_500000_CN_323880677_500000/LConn3 -- bus284/LConn1 -- _CN_232408714_500000_CN_323016571_500000/RConn3
  T_323698983_500000_/LConn1 -- _CN_232408714_500000_CN_323698983_500000/RConn1
  T_323698983_500000_/LConn2 -- _CN_232408714_500000_CN_323698983_500000/RConn2
  _CN_232408714_500000_CN_323698983_500000/RConn3 -- T_323698983_500000_/LConn3 -- bus285/LConn1
  T_323965697_500000_/LConn1 -- _CN_232408714_500000_CN_323965697_500000/RConn1
  T_323965697_500000_/LConn2 -- _CN_232408714_500000_CN_323965697_500000/RConn2
  _CN_232408714_500000_CN_323965697_500000/RConn3 -- T_323965697_500000_/LConn3 -- bus286/LConn1
  T_323880677_500000_/LConn1 -- _CN_232408714_500000_CN_323880677_500000/RConn1
  T_323880677_500000_/LConn2 -- _CN_232408714_500000_CN_323880677_500000/RConn2
  _CN_232408714_500000_CN_323880677_500000/RConn3 -- T_323880677_500000_/LConn3 -- bus287/LConn1
  T_287076644__/LConn1 -- _CN_287088780_500000_CN_287076644_500000/RConn1
  T_287076644__/LConn2 -- _CN_287088780_500000_CN_287076644_500000/RConn2
  _CN_287088780_500000_CN_287076644_500000/RConn3 -- T_287076644__/LConn3 -- bus288/LConn1
  _CN_287088780_500000_CN_287076645_500000/RConn1 -- T_287076645__/LConn1 -- _CN_100600532_500000_CN_287076645_500000/LConn1 -- _CN_287076645_500000_CN_390078007_500000/LConn1
  _CN_287088780_500000_CN_287076645_500000/RConn2 -- T_287076645__/LConn2 -- _CN_100600532_500000_CN_287076645_500000/LConn2 -- _CN_287076645_500000_CN_390078007_500000/LConn2
  _CN_287088780_500000_CN_287076645_500000/RConn3 -- T_287076645__/LConn3 -- _CN_100600532_500000_CN_287076645_500000/LConn3 -- _CN_287076645_500000_CN_390078007_500000/LConn3 -- bus289/LConn1
  T_314351248_500000_/LConn1 -- _CN_314351248_500000_CN_207327989_500000/LConn1
  T_314351248_500000_/LConn2 -- _CN_314351248_500000_CN_207327989_500000/LConn2
  _CN_314351248_500000_CN_207327989_500000/LConn3 -- T_314351248_500000_/LConn3 -- bus290/LConn1
  T_207327989_500000_/LConn1 -- _CN_314351248_500000_CN_207327989_500000/RConn1
  T_207327989_500000_/LConn2 -- _CN_314351248_500000_CN_207327989_500000/RConn2
  _CN_314351248_500000_CN_207327989_500000/RConn3 -- T_207327989_500000_/LConn3 -- bus291/LConn1
  _CN_313934998_500000_CN_178542455_500000/LConn1 -- T_313934998_500000_/LConn1 -- _CN_313934998_500000_CN_313954993_500000/LConn1
  _CN_313934998_500000_CN_178542455_500000/LConn2 -- T_313934998_500000_/LConn2 -- _CN_313934998_500000_CN_313954993_500000/LConn2
  _CN_313934998_500000_CN_178542455_500000/LConn3 -- T_313934998_500000_/LConn3 -- _CN_313934998_500000_CN_313954993_500000/LConn3 -- bus292/LConn1
  T_178542455_500000_/LConn1 -- _CN_313934998_500000_CN_178542455_500000/RConn1
  T_178542455_500000_/LConn2 -- _CN_313934998_500000_CN_178542455_500000/RConn2
  _CN_313934998_500000_CN_178542455_500000/RConn3 -- T_178542455_500000_/LConn3 -- bus293/LConn1
  _CN_313934998_500000_CN_313954993_500000/RConn1 -- T_313954993_500000_/LConn1 -- _CN_313954993_500000_CN_312583866_500000/LConn1
  _CN_313934998_500000_CN_313954993_500000/RConn2 -- T_313954993_500000_/LConn2 -- _CN_313954993_500000_CN_312583866_500000/LConn2
  _CN_313934998_500000_CN_313954993_500000/RConn3 -- T_313954993_500000_/LConn3 -- _CN_313954993_500000_CN_312583866_500000/LConn3 -- bus294/LConn1
  T_157709467__/LConn1 -- _CN_157709467_500000_CN_157709465_500000/LConn1
  T_157709467__/LConn2 -- _CN_157709467_500000_CN_157709465_500000/LConn2
  _CN_157709467_500000_CN_157709465_500000/LConn3 -- T_157709467__/LConn3 -- bus295/LConn1
  G_157709465_Dezhou_power_station/RConn1 -- _CN_157709467_500000_CN_157709465_500000/RConn1
  G_157709465_Dezhou_power_station/RConn2 -- _CN_157709467_500000_CN_157709465_500000/RConn2
  _CN_157709467_500000_CN_157709465_500000/RConn3 -- G_157709465_Dezhou_power_station/RConn3 -- bus296/LConn1
  T_181221620_500000_500KV三汊湾变电站/LConn1 -- _CN_143214751_500000_CN_181221620_500000/RConn1
  T_181221620_500000_500KV三汊湾变电站/LConn2 -- _CN_143214751_500000_CN_181221620_500000/RConn2
  _CN_143214751_500000_CN_181221620_500000/RConn3 -- T_181221620_500000_500KV三汊湾变电站/LConn3 -- bus297/LConn1
  T_276719460__/LConn1 -- 昌平一房山500kV紧_CN_275985691_500000_CN_276719460_500000/RConn1
  T_276719460__/LConn2 -- 昌平一房山500kV紧_CN_275985691_500000_CN_276719460_500000/RConn2
  昌平一房山500kV紧_CN_275985691_500000_CN_276719460_500000/RConn3 -- T_276719460__/LConn3 -- bus298/LConn1
  T_287591085_500000_国家电网500千伏特高压练塘变电站/LConn1 -- _CN_287591085_500000_CN_95805677_500000/LConn1
  T_287591085_500000_国家电网500千伏特高压练塘变电站/LConn2 -- _CN_287591085_500000_CN_95805677_500000/LConn2
  _CN_287591085_500000_CN_95805677_500000/LConn3 -- T_287591085_500000_国家电网500千伏特高压练塘变电站/LConn3 -- bus299/LConn1
  _CN_287591085_500000_CN_95805677_500000/RConn1 -- T_95805677_500000_/LConn1 -- _CN_95805677_500000_CN_286137154_500000/LConn1 -- _CN_95805677_500000_CN_106027291_500000/LConn1
  _CN_287591085_500000_CN_95805677_500000/RConn2 -- T_95805677_500000_/LConn2 -- _CN_95805677_500000_CN_286137154_500000/LConn2 -- _CN_95805677_500000_CN_106027291_500000/LConn2
  _CN_287591085_500000_CN_95805677_500000/RConn3 -- T_95805677_500000_/LConn3 -- _CN_95805677_500000_CN_286137154_500000/LConn3 -- _CN_95805677_500000_CN_106027291_500000/LConn3 -- bus300/LConn1
  T_128727214__/LConn1 -- _CN_128727214_500000_CN_171491186_500000/LConn1
  T_128727214__/LConn2 -- _CN_128727214_500000_CN_171491186_500000/LConn2
  _CN_128727214_500000_CN_171491186_500000/LConn3 -- T_128727214__/LConn3 -- bus301/LConn1
  T_171491186__/LConn1 -- _CN_128727214_500000_CN_171491186_500000/RConn1
  T_171491186__/LConn2 -- _CN_128727214_500000_CN_171491186_500000/RConn2
  _CN_128727214_500000_CN_171491186_500000/RConn3 -- T_171491186__/LConn3 -- bus302/LConn1
  _CN_313954993_500000_CN_312583866_500000/RConn1 -- T_312583866_500000_/LConn1 -- _CN_312583866_500000_CN_254904701_500000/LConn1
  _CN_313954993_500000_CN_312583866_500000/RConn2 -- T_312583866_500000_/LConn2 -- _CN_312583866_500000_CN_254904701_500000/LConn2
  _CN_313954993_500000_CN_312583866_500000/RConn3 -- T_312583866_500000_/LConn3 -- _CN_312583866_500000_CN_254904701_500000/LConn3 -- bus303/LConn1
  T_315071509_500000_/LConn1 -- _CN_315071509_500000_CN_315071478_500000/LConn1
  T_315071509_500000_/LConn2 -- _CN_315071509_500000_CN_315071478_500000/LConn2
  _CN_315071509_500000_CN_315071478_500000/LConn3 -- T_315071509_500000_/LConn3 -- bus304/LConn1
  T_315071478_500000_/LConn1 -- _CN_315071509_500000_CN_315071478_500000/RConn1
  T_315071478_500000_/LConn2 -- _CN_315071509_500000_CN_315071478_500000/RConn2
  _CN_315071509_500000_CN_315071478_500000/RConn3 -- T_315071478_500000_/LConn3 -- bus305/LConn1
  T_254904701_500000_/LConn1 -- _CN_312583866_500000_CN_254904701_500000/RConn1
  T_254904701_500000_/LConn2 -- _CN_312583866_500000_CN_254904701_500000/RConn2
  _CN_312583866_500000_CN_254904701_500000/RConn3 -- T_254904701_500000_/LConn3 -- bus306/LConn1
  T_79198909_500000_/LConn1 -- _CN_79198909_500000_CN_135466215_500000/LConn1
  T_79198909_500000_/LConn2 -- _CN_79198909_500000_CN_135466215_500000/LConn2
  _CN_79198909_500000_CN_135466215_500000/LConn3 -- T_79198909_500000_/LConn3 -- bus307/LConn1
  _CN_79198909_500000_CN_135466215_500000/RConn1 -- T_135466215_500000_天津北郊/LConn1 -- _CN_135466215_500000_CN_312852542_500000/RConn1 -- _CN_135466215_500000_CN_221891107_500000/RConn1
  _CN_79198909_500000_CN_135466215_500000/RConn2 -- T_135466215_500000_天津北郊/LConn2 -- _CN_135466215_500000_CN_312852542_500000/RConn2 -- _CN_135466215_500000_CN_221891107_500000/RConn2
  _CN_79198909_500000_CN_135466215_500000/RConn3 -- T_135466215_500000_天津北郊/LConn3 -- _CN_135466215_500000_CN_312852542_500000/RConn3 -- bus308/LConn1 -- _CN_135466215_500000_CN_221891107_500000/RConn3
  T_312922832_500000_/LConn1 -- _CN_312922832_500000_CN_146077915_500000/RConn1
  T_312922832_500000_/LConn2 -- _CN_312922832_500000_CN_146077915_500000/RConn2
  _CN_312922832_500000_CN_146077915_500000/RConn3 -- T_312922832_500000_/LConn3 -- bus309/LConn1
  _CN_281631607_500000_CN_163357534_500000/RConn1 -- T_163357534__/LConn1 -- _CN_163357515_500000_CN_163357534_500000/LConn1 -- _CN_166670597_500000_CN_163357534_500000/LConn1
  _CN_281631607_500000_CN_163357534_500000/RConn2 -- T_163357534__/LConn2 -- _CN_163357515_500000_CN_163357534_500000/LConn2 -- _CN_166670597_500000_CN_163357534_500000/LConn2
  _CN_281631607_500000_CN_163357534_500000/RConn3 -- T_163357534__/LConn3 -- _CN_163357515_500000_CN_163357534_500000/LConn3 -- bus310/LConn1 -- _CN_166670597_500000_CN_163357534_500000/LConn3
  _CN_100600532_500000_CN_287076645_500000/RConn1 -- T_100600532__/LConn1 -- _CN_100600532_500000_CN_106027291_500000/LConn1 -- _CN_100600532_500000_CN_163021047_500000/LConn1 -- _CN_100600532_500000_CN_286930852_500000/LConn1 -- _CN_100600532_500000_CN_283658124_500000/LConn1
  _CN_100600532_500000_CN_287076645_500000/RConn2 -- T_100600532__/LConn2 -- _CN_100600532_500000_CN_106027291_500000/LConn2 -- _CN_100600532_500000_CN_163021047_500000/LConn2 -- _CN_100600532_500000_CN_286930852_500000/LConn2 -- _CN_100600532_500000_CN_283658124_500000/LConn2
  _CN_100600532_500000_CN_287076645_500000/RConn3 -- T_100600532__/LConn3 -- _CN_100600532_500000_CN_106027291_500000/LConn3 -- bus311/LConn1 -- _CN_100600532_500000_CN_163021047_500000/LConn3 -- _CN_100600532_500000_CN_286930852_500000/LConn3 -- _CN_100600532_500000_CN_283658124_500000/LConn3
  _CN_100600532_500000_CN_163021047_500000/RConn1 -- T_163021047__/LConn1 -- _CN_163021047_500000_CN_163357515_500000/LConn1
  _CN_100600532_500000_CN_163021047_500000/RConn2 -- T_163021047__/LConn2 -- _CN_163021047_500000_CN_163357515_500000/LConn2
  _CN_100600532_500000_CN_163021047_500000/RConn3 -- T_163021047__/LConn3 -- _CN_163021047_500000_CN_163357515_500000/LConn3 -- bus312/LConn1
  T_286930852__/LConn1 -- _CN_100600532_500000_CN_286930852_500000/RConn1
  T_286930852__/LConn2 -- _CN_100600532_500000_CN_286930852_500000/RConn2
  _CN_100600532_500000_CN_286930852_500000/RConn3 -- T_286930852__/LConn3 -- bus313/LConn1
  _CN_100600532_500000_CN_283658124_500000/RConn1 -- T_283658124__/LConn1 -- _CN_170703096_500000_CN_283658124_500000/LConn1
  _CN_100600532_500000_CN_283658124_500000/RConn2 -- T_283658124__/LConn2 -- _CN_170703096_500000_CN_283658124_500000/LConn2
  _CN_100600532_500000_CN_283658124_500000/RConn3 -- T_283658124__/LConn3 -- _CN_170703096_500000_CN_283658124_500000/LConn3 -- bus314/LConn1
  _CN_100600532_500000_CN_106027291_500000/RConn1 -- T_106027291_500000_/LConn1 -- _CN_95805677_500000_CN_106027291_500000/RConn1
  _CN_100600532_500000_CN_106027291_500000/RConn2 -- T_106027291_500000_/LConn2 -- _CN_95805677_500000_CN_106027291_500000/RConn2
  _CN_100600532_500000_CN_106027291_500000/RConn3 -- T_106027291_500000_/LConn3 -- _CN_95805677_500000_CN_106027291_500000/RConn3 -- bus315/LConn1
  T_334707427__/LConn1 -- _CN_334707427_500000_CN_167981876_500000/LConn1
  T_334707427__/LConn2 -- _CN_334707427_500000_CN_167981876_500000/LConn2
  _CN_334707427_500000_CN_167981876_500000/LConn3 -- T_334707427__/LConn3 -- bus316/LConn1
  _CN_334707427_500000_CN_167981876_500000/RConn1 -- T_167981876_500000_/LConn1 -- _CN_167981876_500000_CN_321690480_500000/LConn1 -- _CN_167981876_500000_CN_315071484_500000/LConn1
  _CN_334707427_500000_CN_167981876_500000/RConn2 -- T_167981876_500000_/LConn2 -- _CN_167981876_500000_CN_321690480_500000/LConn2 -- _CN_167981876_500000_CN_315071484_500000/LConn2
  _CN_334707427_500000_CN_167981876_500000/RConn3 -- T_167981876_500000_/LConn3 -- _CN_167981876_500000_CN_321690480_500000/LConn3 -- bus317/LConn1 -- _CN_167981876_500000_CN_315071484_500000/LConn3
  T_286137154__/LConn1 -- _CN_95805677_500000_CN_286137154_500000/RConn1
  T_286137154__/LConn2 -- _CN_95805677_500000_CN_286137154_500000/RConn2
  _CN_95805677_500000_CN_286137154_500000/RConn3 -- T_286137154__/LConn3 -- bus318/LConn1
  T_303677167__/LConn1 -- _CN_303677167_500000_CN_314288467_500000/LConn1
  T_303677167__/LConn2 -- _CN_303677167_500000_CN_314288467_500000/LConn2
  _CN_303677167_500000_CN_314288467_500000/LConn3 -- T_303677167__/LConn3 -- bus319/LConn1
  _CN_303677167_500000_CN_314288467_500000/RConn1 -- T_314288467_500000_/LConn1 -- _CN_314288467_500000_CN_314164572_500000/LConn1
  _CN_303677167_500000_CN_314288467_500000/RConn2 -- T_314288467_500000_/LConn2 -- _CN_314288467_500000_CN_314164572_500000/LConn2
  _CN_303677167_500000_CN_314288467_500000/RConn3 -- T_314288467_500000_/LConn3 -- _CN_314288467_500000_CN_314164572_500000/LConn3 -- bus320/LConn1
  _CN_163021047_500000_CN_163357515_500000/RConn1 -- T_163357515__/LConn1 -- _CN_163357508_500000_CN_163357515_500000/LConn1 -- _CN_163357515_500000_CN_163357534_500000/RConn1
  _CN_163021047_500000_CN_163357515_500000/RConn2 -- T_163357515__/LConn2 -- _CN_163357508_500000_CN_163357515_500000/LConn2 -- _CN_163357515_500000_CN_163357534_500000/RConn2
  _CN_163021047_500000_CN_163357515_500000/RConn3 -- T_163357515__/LConn3 -- _CN_163357508_500000_CN_163357515_500000/LConn3 -- _CN_163357515_500000_CN_163357534_500000/RConn3 -- bus321/LConn1
  _CN_170703096_500000_CN_166670597_500000/LConn1 -- T_170703096_500000_/LConn1 -- _CN_170703096_500000_CN_283658124_500000/RConn1 -- _CN_170703096_500000_CN_283658133_500000/LConn1 -- _CN_170703096_500000_CN_283658134_500000/LConn1
  _CN_170703096_500000_CN_166670597_500000/LConn2 -- T_170703096_500000_/LConn2 -- _CN_170703096_500000_CN_283658124_500000/RConn2 -- _CN_170703096_500000_CN_283658133_500000/LConn2 -- _CN_170703096_500000_CN_283658134_500000/LConn2
  _CN_170703096_500000_CN_166670597_500000/LConn3 -- T_170703096_500000_/LConn3 -- _CN_170703096_500000_CN_283658124_500000/RConn3 -- _CN_170703096_500000_CN_283658133_500000/LConn3 -- bus322/LConn1 -- _CN_170703096_500000_CN_283658134_500000/LConn3
  _CN_170703096_500000_CN_166670597_500000/RConn1 -- T_166670597__/LConn1 -- _CN_166670597_500000_CN_163357534_500000/RConn1 -- _CN_166670597_500000_CN_166670647_220000/RConn1
  _CN_170703096_500000_CN_166670597_500000/RConn2 -- T_166670597__/LConn2 -- _CN_166670597_500000_CN_163357534_500000/RConn2 -- _CN_166670597_500000_CN_166670647_220000/RConn2
  _CN_170703096_500000_CN_166670597_500000/RConn3 -- T_166670597__/LConn3 -- _CN_166670597_500000_CN_163357534_500000/RConn3 -- _CN_166670597_500000_CN_166670647_220000/RConn3 -- bus323/LConn1
  T_283658134__/LConn1 -- _CN_170703096_500000_CN_283658134_500000/RConn1
  T_283658134__/LConn2 -- _CN_170703096_500000_CN_283658134_500000/RConn2
  _CN_170703096_500000_CN_283658134_500000/RConn3 -- T_283658134__/LConn3 -- bus324/LConn1
  _CN_170703096_500000_CN_283658133_500000/RConn1 -- T_283658133__/LConn1 -- _CN_283658133_500000_CN_121056862_220000/RConn1
  _CN_170703096_500000_CN_283658133_500000/RConn2 -- T_283658133__/LConn2 -- _CN_283658133_500000_CN_121056862_220000/RConn2
  _CN_170703096_500000_CN_283658133_500000/RConn3 -- T_283658133__/LConn3 -- _CN_283658133_500000_CN_121056862_220000/RConn3 -- bus325/LConn1
  T_300336767__/LConn1 -- _CN_300336767_500000_CN_301061895_500000/LConn1
  T_300336767__/LConn2 -- _CN_300336767_500000_CN_301061895_500000/LConn2
  _CN_300336767_500000_CN_301061895_500000/LConn3 -- T_300336767__/LConn3 -- bus326/LConn1
  T_301061895__/LConn1 -- _CN_300336767_500000_CN_301061895_500000/RConn1
  T_301061895__/LConn2 -- _CN_300336767_500000_CN_301061895_500000/RConn2
  _CN_300336767_500000_CN_301061895_500000/RConn3 -- T_301061895__/LConn3 -- bus327/LConn1
  T_327908612_500000_/LConn1 -- _CN_327908612_500000_CN_220524234_500000/LConn1
  T_327908612_500000_/LConn2 -- _CN_327908612_500000_CN_220524234_500000/LConn2
  _CN_327908612_500000_CN_220524234_500000/LConn3 -- T_327908612_500000_/LConn3 -- bus328/LConn1
  G_220524234_/RConn1 -- _CN_327908612_500000_CN_220524234_500000/RConn1
  G_220524234_/RConn2 -- _CN_327908612_500000_CN_220524234_500000/RConn2
  _CN_327908612_500000_CN_220524234_500000/RConn3 -- G_220524234_/RConn3 -- bus329/LConn1
  _CN_424682265_500000_CN_323016571_500000/RConn1 -- T_424682265__/LConn1 -- _CN_424682265_500000_CN_323032986_500000/LConn1
  _CN_424682265_500000_CN_323016571_500000/RConn2 -- T_424682265__/LConn2 -- _CN_424682265_500000_CN_323032986_500000/LConn2
  _CN_424682265_500000_CN_323016571_500000/RConn3 -- T_424682265__/LConn3 -- _CN_424682265_500000_CN_323032986_500000/LConn3 -- bus330/LConn1
  T_323032986__/LConn1 -- _CN_424682265_500000_CN_323032986_500000/RConn1
  T_323032986__/LConn2 -- _CN_424682265_500000_CN_323032986_500000/RConn2
  _CN_424682265_500000_CN_323032986_500000/RConn3 -- T_323032986__/LConn3 -- bus331/LConn1
  T_424682272__/LConn1 -- _CN_151766812_500000_CN_424682272_500000/RConn1
  T_424682272__/LConn2 -- _CN_151766812_500000_CN_424682272_500000/RConn2
  _CN_151766812_500000_CN_424682272_500000/RConn3 -- T_424682272__/LConn3 -- bus332/LConn1
  _CN_287076645_500000_CN_390078007_500000/RConn1 -- G_390078007_/RConn1 -- _CN_287200191_500000_CN_390078007_500000/LConn1
  _CN_287076645_500000_CN_390078007_500000/RConn2 -- G_390078007_/RConn2 -- _CN_287200191_500000_CN_390078007_500000/LConn2
  _CN_287076645_500000_CN_390078007_500000/RConn3 -- G_390078007_/RConn3 -- _CN_287200191_500000_CN_390078007_500000/LConn3 -- bus333/LConn1
  T_315071484_500000_/LConn1 -- _CN_167981876_500000_CN_315071484_500000/RConn1
  T_315071484_500000_/LConn2 -- _CN_167981876_500000_CN_315071484_500000/RConn2
  _CN_167981876_500000_CN_315071484_500000/RConn3 -- T_315071484_500000_/LConn3 -- bus334/LConn1
  _CN_167981876_500000_CN_321690480_500000/RConn1 -- T_321690480_500000_/LConn1 -- _CN_321690463_500000_CN_321690480_500000/LConn1
  _CN_167981876_500000_CN_321690480_500000/RConn2 -- T_321690480_500000_/LConn2 -- _CN_321690463_500000_CN_321690480_500000/LConn2
  _CN_167981876_500000_CN_321690480_500000/RConn3 -- T_321690480_500000_/LConn3 -- _CN_321690463_500000_CN_321690480_500000/LConn3 -- bus335/LConn1
  T_132430137_500000_/LConn1 -- _CN_132430137_500000_CN_132503439_500000/LConn1
  T_132430137_500000_/LConn2 -- _CN_132430137_500000_CN_132503439_500000/LConn2
  _CN_132430137_500000_CN_132503439_500000/LConn3 -- T_132430137_500000_/LConn3 -- bus336/LConn1
  T_132503439_220000_/LConn1 -- _CN_132430137_500000_CN_132503439_500000/RConn1
  T_132503439_220000_/LConn2 -- _CN_132430137_500000_CN_132503439_500000/RConn2
  _CN_132430137_500000_CN_132503439_500000/RConn3 -- T_132503439_220000_/LConn3 -- bus337/LConn1
  T_163357508__Zhengping_Static_Inverter_Plant/LConn1 -- _CN_163357508_500000_CN_163357515_500000/RConn1
  T_163357508__Zhengping_Static_Inverter_Plant/LConn2 -- _CN_163357508_500000_CN_163357515_500000/RConn2
  _CN_163357508_500000_CN_163357515_500000/RConn3 -- T_163357508__Zhengping_Static_Inverter_Plant/LConn3 -- bus338/LConn1
  G_251522340_/RConn1 -- _CN_251393861_500000_CN_251522340_500000/RConn1
  G_251522340_/RConn2 -- _CN_251393861_500000_CN_251522340_500000/RConn2
  _CN_251393861_500000_CN_251522340_500000/RConn3 -- G_251522340_/RConn3 -- bus339/LConn1
  T_314164572_500000_/LConn1 -- _CN_314288467_500000_CN_314164572_500000/RConn1
  T_314164572_500000_/LConn2 -- _CN_314288467_500000_CN_314164572_500000/RConn2
  _CN_314288467_500000_CN_314164572_500000/RConn3 -- T_314164572_500000_/LConn3 -- bus340/LConn1
  T_321690463_500000_/LConn1 -- _CN_321690463_500000_CN_321690480_500000/RConn1
  T_321690463_500000_/LConn2 -- _CN_321690463_500000_CN_321690480_500000/RConn2
  _CN_321690463_500000_CN_321690480_500000/RConn3 -- T_321690463_500000_/LConn3 -- bus341/LConn1
  G_171491178_/RConn1 -- _CN_171491177_500000_CN_171491178_500000/RConn1
  G_171491178_/RConn2 -- _CN_171491177_500000_CN_171491178_500000/RConn2
  _CN_171491177_500000_CN_171491178_500000/RConn3 -- G_171491178_/RConn3 -- bus342/LConn1
  T_147708063_500000_/LConn1 -- _CN_188829044_500000_CN_147708063_500000/RConn1
  T_147708063_500000_/LConn2 -- _CN_188829044_500000_CN_147708063_500000/RConn2
  _CN_188829044_500000_CN_147708063_500000/RConn3 -- T_147708063_500000_/LConn3 -- bus343/LConn1
  _CN_277499262_500000_CN_312852542_500000/RConn1 -- T_277499262__/LConn1 -- _CN_277499262_500000_CN_221891107_500000/RConn1
  _CN_277499262_500000_CN_312852542_500000/RConn2 -- T_277499262__/LConn2 -- _CN_277499262_500000_CN_221891107_500000/RConn2
  _CN_277499262_500000_CN_312852542_500000/RConn3 -- T_277499262__/LConn3 -- _CN_277499262_500000_CN_221891107_500000/RConn3 -- bus344/LConn1
  T_181090227_500000;220000_/LConn1 -- _CN_327333768_500000_CN_181090227_500000/RConn1
  T_181090227_500000;220000_/LConn2 -- _CN_327333768_500000_CN_181090227_500000/RConn2
  _CN_327333768_500000_CN_181090227_500000/RConn3 -- T_181090227_500000;220000_/LConn3 -- bus345/LConn1
  T_312925118_500000_/LConn1 -- _CN_312925118_500000_CN_314606532_500000/LConn1
  T_312925118_500000_/LConn2 -- _CN_312925118_500000_CN_314606532_500000/LConn2
  _CN_312925118_500000_CN_314606532_500000/LConn3 -- T_312925118_500000_/LConn3 -- bus346/LConn1
  T_314606532_500000_/LConn1 -- _CN_312925118_500000_CN_314606532_500000/RConn1
  T_314606532_500000_/LConn2 -- _CN_312925118_500000_CN_314606532_500000/RConn2
  _CN_312925118_500000_CN_314606532_500000/RConn3 -- T_314606532_500000_/LConn3 -- bus347/LConn1
  T_287200191__/LConn1 -- _CN_287200191_500000_CN_390078007_500000/RConn1
  T_287200191__/LConn2 -- _CN_287200191_500000_CN_390078007_500000/RConn2
  _CN_287200191_500000_CN_390078007_500000/RConn3 -- T_287200191__/LConn3 -- bus348/LConn1
  T_121056846__/RConn1 -- L_121056846/LConn1
  T_121056846__/RConn2 -- L_121056846/LConn2
  L_121056846/LConn3 -- T_121056846__/RConn3 -- bus349/LConn1
  T_347775701_110000_110kV根亲变电站/RConn1 -- L_347775701/LConn1
  T_347775701_110000_110kV根亲变电站/RConn2 -- L_347775701/LConn2
  L_347775701/LConn3 -- T_347775701_110000_110kV根亲变电站/RConn3 -- bus350/LConn1
  T_177340388_110000_杜营110KV变电站/RConn1 -- L_177340388/LConn1
  T_177340388_110000_杜营110KV变电站/RConn2 -- L_177340388/LConn2
  L_177340388/LConn3 -- T_177340388_110000_杜营110KV变电站/RConn3 -- bus351/LConn1
  T_265301080_110000_/RConn1 -- L_265301080/LConn1
  T_265301080_110000_/RConn2 -- L_265301080/LConn2
  L_265301080/LConn3 -- T_265301080_110000_/RConn3 -- bus352/LConn1
  T_145499354__/RConn1 -- L_145499354/LConn1
  T_145499354__/RConn2 -- L_145499354/LConn2
  L_145499354/LConn3 -- T_145499354__/RConn3 -- bus353/LConn1
  T_145499355__/RConn1 -- L_145499355/LConn1
  T_145499355__/RConn2 -- L_145499355/LConn2
  L_145499355/LConn3 -- T_145499355__/RConn3 -- bus354/LConn1
  T_145499356__/RConn1 -- L_145499356/LConn1
  T_145499356__/RConn2 -- L_145499356/LConn2
  L_145499356/LConn3 -- T_145499356__/RConn3 -- bus355/LConn1
  T_255311431__/RConn1 -- L_255311431/LConn1
  T_255311431__/RConn2 -- L_255311431/LConn2
  L_255311431/LConn3 -- T_255311431__/RConn3 -- bus356/LConn1
  T_161577477_220000_/RConn1 -- L_161577477/LConn1
  T_161577477_220000_/RConn2 -- L_161577477/LConn2
  L_161577477/LConn3 -- T_161577477_220000_/RConn3 -- bus357/LConn1
  T_278169207__/RConn1 -- L_278169207/LConn1
  T_278169207__/RConn2 -- L_278169207/LConn2
  L_278169207/LConn3 -- T_278169207__/RConn3 -- bus358/LConn1
  T_313629190_220000_/RConn1 -- L_313629190/LConn1
  T_313629190_220000_/RConn2 -- L_313629190/LConn2
  L_313629190/LConn3 -- T_313629190_220000_/RConn3 -- bus359/LConn1
  T_315269978_220000_/RConn1 -- L_315269978/LConn1
  T_315269978_220000_/RConn2 -- L_315269978/LConn2
  L_315269978/LConn3 -- T_315269978_220000_/RConn3 -- bus360/LConn1
  T_328842159_220000_/RConn1 -- L_328842159/LConn1
  T_328842159_220000_/RConn2 -- L_328842159/LConn2
  L_328842159/LConn3 -- T_328842159_220000_/RConn3 -- bus361/LConn1
  T_284083287__/RConn1 -- L_284083287/LConn1
  T_284083287__/RConn2 -- L_284083287/LConn2
  L_284083287/LConn3 -- T_284083287__/RConn3 -- bus362/LConn1
  T_284083294__/RConn1 -- L_284083294/LConn1
  T_284083294__/RConn2 -- L_284083294/LConn2
  L_284083294/LConn3 -- T_284083294__/RConn3 -- bus363/LConn1
  T_284083280__/RConn1 -- L_284083280/LConn1
  T_284083280__/RConn2 -- L_284083280/LConn2
  L_284083280/LConn3 -- T_284083280__/RConn3 -- bus364/LConn1
  T_315204024_220000_/RConn1 -- L_315204024/LConn1
  T_315204024_220000_/RConn2 -- L_315204024/LConn2
  L_315204024/LConn3 -- T_315204024_220000_/RConn3 -- bus365/LConn1
  T_150403605_220000_/RConn1 -- L_150403605/LConn1
  T_150403605_220000_/RConn2 -- L_150403605/LConn2
  L_150403605/LConn3 -- T_150403605_220000_/RConn3 -- bus366/LConn1
  T_355642647__/RConn1 -- L_355642647/LConn1
  T_355642647__/RConn2 -- L_355642647/LConn2
  L_355642647/LConn3 -- T_355642647__/RConn3 -- bus367/LConn1
  T_95783449__/RConn1 -- L_95783449/LConn1
  T_95783449__/RConn2 -- L_95783449/LConn2
  L_95783449/LConn3 -- T_95783449__/RConn3 -- bus368/LConn1
  T_104955669__/RConn1 -- L_104955669/LConn1
  T_104955669__/RConn2 -- L_104955669/LConn2
  L_104955669/LConn3 -- T_104955669__/RConn3 -- bus369/LConn1
  T_279415839__/RConn1 -- L_279415839/LConn1
  T_279415839__/RConn2 -- L_279415839/LConn2
  L_279415839/LConn3 -- T_279415839__/RConn3 -- bus370/LConn1
  T_279415840__/RConn1 -- L_279415840/LConn1
  T_279415840__/RConn2 -- L_279415840/LConn2
  L_279415840/LConn3 -- T_279415840__/RConn3 -- bus371/LConn1
  T_201197023_220000_/RConn1 -- L_201197023/LConn1
  T_201197023_220000_/RConn2 -- L_201197023/LConn2
  L_201197023/LConn3 -- T_201197023_220000_/RConn3 -- bus372/LConn1
  T_275706404__/RConn1 -- L_275706404/LConn1
  T_275706404__/RConn2 -- L_275706404/LConn2
  L_275706404/LConn3 -- T_275706404__/RConn3 -- bus373/LConn1
  T_276589707__/RConn1 -- L_276589707/LConn1
  T_276589707__/RConn2 -- L_276589707/LConn2
  L_276589707/LConn3 -- T_276589707__/RConn3 -- bus374/LConn1
  T_119206438_220000_/RConn1 -- L_119206438/LConn1
  T_119206438_220000_/RConn2 -- L_119206438/LConn2
  L_119206438/LConn3 -- T_119206438_220000_/RConn3 -- bus375/LConn1
  T_119206440_220000_/RConn1 -- L_119206440/LConn1
  T_119206440_220000_/RConn2 -- L_119206440/LConn2
  L_119206440/LConn3 -- T_119206440_220000_/RConn3 -- bus376/LConn1
  T_223806191_220000_/RConn1 -- L_223806191/LConn1
  T_223806191_220000_/RConn2 -- L_223806191/LConn2
  L_223806191/LConn3 -- T_223806191_220000_/RConn3 -- bus377/LConn1
  T_279419433__/RConn1 -- L_279419433/LConn1
  T_279419433__/RConn2 -- L_279419433/LConn2
  L_279419433/LConn3 -- T_279419433__/RConn3 -- bus378/LConn1
  T_162378077__/RConn1 -- L_162378077/LConn1
  T_162378077__/RConn2 -- L_162378077/LConn2
  L_162378077/LConn3 -- T_162378077__/RConn3 -- bus379/LConn1
  T_162378099__/RConn1 -- L_162378099/LConn1
  T_162378099__/RConn2 -- L_162378099/LConn2
  L_162378099/LConn3 -- T_162378099__/RConn3 -- bus380/LConn1
  T_285846074__/RConn1 -- L_285846074/LConn1
  T_285846074__/RConn2 -- L_285846074/LConn2
  L_285846074/LConn3 -- T_285846074__/RConn3 -- bus381/LConn1
  T_107025759_220000_/RConn1 -- L_107025759/LConn1
  T_107025759_220000_/RConn2 -- L_107025759/LConn2
  L_107025759/LConn3 -- T_107025759_220000_/RConn3 -- bus382/LConn1
  T_330370369__/RConn1 -- L_330370369/LConn1
  T_330370369__/RConn2 -- L_330370369/LConn2
  L_330370369/LConn3 -- T_330370369__/RConn3 -- bus383/LConn1
  T_95783487__/RConn1 -- L_95783487/LConn1
  T_95783487__/RConn2 -- L_95783487/LConn2
  L_95783487/LConn3 -- T_95783487__/RConn3 -- bus384/LConn1
  T_95783492__/RConn1 -- L_95783492/LConn1
  T_95783492__/RConn2 -- L_95783492/LConn2
  L_95783492/LConn3 -- T_95783492__/RConn3 -- bus385/LConn1
  T_284039744__/RConn1 -- L_284039744/LConn1
  T_284039744__/RConn2 -- L_284039744/LConn2
  L_284039744/LConn3 -- T_284039744__/RConn3 -- bus386/LConn1
  T_188973331_220000_/RConn1 -- L_188973331/LConn1
  T_188973331_220000_/RConn2 -- L_188973331/LConn2
  L_188973331/LConn3 -- T_188973331_220000_/RConn3 -- bus387/LConn1
  T_95093839__/RConn1 -- L_95093839/LConn1
  T_95093839__/RConn2 -- L_95093839/LConn2
  L_95093839/LConn3 -- T_95093839__/RConn3 -- bus388/LConn1
  T_95783495__/RConn1 -- L_95783495/LConn1
  T_95783495__/RConn2 -- L_95783495/LConn2
  L_95783495/LConn3 -- T_95783495__/RConn3 -- bus389/LConn1
  T_95513512__/RConn1 -- L_95513512/LConn1
  T_95513512__/RConn2 -- L_95513512/LConn2
  L_95513512/LConn3 -- T_95513512__/RConn3 -- bus390/LConn1
  T_255311430__/RConn1 -- L_255311430/LConn1
  T_255311430__/RConn2 -- L_255311430/LConn2
  L_255311430/LConn3 -- T_255311430__/RConn3 -- bus391/LConn1
  T_95783496__/RConn1 -- L_95783496/LConn1
  T_95783496__/RConn2 -- L_95783496/LConn2
  L_95783496/LConn3 -- T_95783496__/RConn3 -- bus392/LConn1
  T_284083277__/RConn1 -- L_284083277/LConn1
  T_284083277__/RConn2 -- L_284083277/LConn2
  L_284083277/LConn3 -- T_284083277__/RConn3 -- bus393/LConn1
  T_284083293__/RConn1 -- L_284083293/LConn1
  T_284083293__/RConn2 -- L_284083293/LConn2
  L_284083293/LConn3 -- T_284083293__/RConn3 -- bus394/LConn1
  T_225119562__/RConn1 -- L_225119562/LConn1
  T_225119562__/RConn2 -- L_225119562/LConn2
  L_225119562/LConn3 -- T_225119562__/RConn3 -- bus395/LConn1
  T_314606534_220000_/RConn1 -- L_314606534/LConn1
  T_314606534_220000_/RConn2 -- L_314606534/LConn2
  L_314606534/LConn3 -- T_314606534_220000_/RConn3 -- bus396/LConn1
  T_147710033_220000_/RConn1 -- L_147710033/LConn1
  T_147710033_220000_/RConn2 -- L_147710033/LConn2
  L_147710033/LConn3 -- T_147710033_220000_/RConn3 -- bus397/LConn1
  T_280851769__/RConn1 -- L_280851769/LConn1
  T_280851769__/RConn2 -- L_280851769/LConn2
  L_280851769/LConn3 -- T_280851769__/RConn3 -- bus398/LConn1
  T_323016549_500000_/RConn1 -- L_323016549/LConn1
  T_323016549_500000_/RConn2 -- L_323016549/LConn2
  L_323016549/LConn3 -- T_323016549_500000_/RConn3 -- bus399/LConn1
  T_128731546__/RConn1 -- L_128731546/LConn1
  T_128731546__/RConn2 -- L_128731546/LConn2
  L_128731546/LConn3 -- T_128731546__/RConn3 -- bus400/LConn1
  T_171484817__/RConn1 -- L_171484817/LConn1
  T_171484817__/RConn2 -- L_171484817/LConn2
  L_171484817/LConn3 -- T_171484817__/RConn3 -- bus401/LConn1
  T_170221358_220000_/RConn1 -- L_170221358/LConn1
  T_170221358_220000_/RConn2 -- L_170221358/LConn2
  L_170221358/LConn3 -- T_170221358_220000_/RConn3 -- bus402/LConn1
  T_170206555_500000_Pengzhou_Substation/RConn1 -- L_170206555/LConn1
  T_170206555_500000_Pengzhou_Substation/RConn2 -- L_170206555/LConn2
  L_170206555/LConn3 -- T_170206555_500000_Pengzhou_Substation/RConn3 -- bus403/LConn1
  T_328639863__/RConn1 -- L_328639863/LConn1
  T_328639863__/RConn2 -- L_328639863/LConn2
  L_328639863/LConn3 -- T_328639863__/RConn3 -- bus404/LConn1
  T_313585532_220000_/RConn1 -- L_313585532/LConn1
  T_313585532_220000_/RConn2 -- L_313585532/LConn2
  L_313585532/LConn3 -- T_313585532_220000_/RConn3 -- bus405/LConn1
  T_312852588__/RConn1 -- L_312852588/LConn1
  T_312852588__/RConn2 -- L_312852588/LConn2
  L_312852588/LConn3 -- T_312852588__/RConn3 -- bus406/LConn1
  T_312852605__/RConn1 -- L_312852605/LConn1
  T_312852605__/RConn2 -- L_312852605/LConn2
  L_312852605/LConn3 -- T_312852605__/RConn3 -- bus407/LConn1
  T_279595711__/RConn1 -- L_279595711/LConn1
  T_279595711__/RConn2 -- L_279595711/LConn2
  L_279595711/LConn3 -- T_279595711__/RConn3 -- bus408/LConn1
  T_278530118__/RConn1 -- L_278530118/LConn1
  T_278530118__/RConn2 -- L_278530118/LConn2
  L_278530118/LConn3 -- T_278530118__/RConn3 -- bus409/LConn1
  T_189931119__/RConn1 -- L_189931119/LConn1
  T_189931119__/RConn2 -- L_189931119/LConn2
  L_189931119/LConn3 -- T_189931119__/RConn3 -- bus410/LConn1
  T_319534355__/RConn1 -- L_319534355/LConn1
  T_319534355__/RConn2 -- L_319534355/LConn2
  L_319534355/LConn3 -- T_319534355__/RConn3 -- bus411/LConn1
  T_365846132__/RConn1 -- L_365846132/LConn1
  T_365846132__/RConn2 -- L_365846132/LConn2
  L_365846132/LConn3 -- T_365846132__/RConn3 -- bus412/LConn1
  T_277880965__/RConn1 -- L_277880965/LConn1
  T_277880965__/RConn2 -- L_277880965/LConn2
  L_277880965/LConn3 -- T_277880965__/RConn3 -- bus413/LConn1
  T_264823742_220000_/RConn1 -- L_264823742/LConn1
  T_264823742_220000_/RConn2 -- L_264823742/LConn2
  L_264823742/LConn3 -- T_264823742_220000_/RConn3 -- bus414/LConn1
  T_282759079__/RConn1 -- L_282759079/LConn1
  T_282759079__/RConn2 -- L_282759079/LConn2
  L_282759079/LConn3 -- T_282759079__/RConn3 -- bus415/LConn1
  T_284477051__/RConn1 -- L_284477051/LConn1
  T_284477051__/RConn2 -- L_284477051/LConn2
  L_284477051/LConn3 -- T_284477051__/RConn3 -- bus416/LConn1
  T_312852604__/RConn1 -- L_312852604/LConn1
  T_312852604__/RConn2 -- L_312852604/LConn2
  L_312852604/LConn3 -- T_312852604__/RConn3 -- bus417/LConn1
  T_278062434__/RConn1 -- L_278062434/LConn1
  T_278062434__/RConn2 -- L_278062434/LConn2
  L_278062434/LConn3 -- T_278062434__/RConn3 -- bus418/LConn1
  T_277704920_220000_/RConn1 -- L_277704920/LConn1
  T_277704920_220000_/RConn2 -- L_277704920/LConn2
  L_277704920/LConn3 -- T_277704920_220000_/RConn3 -- bus419/LConn1
  T_147706495_220000_/RConn1 -- L_147706495/LConn1
  T_147706495_220000_/RConn2 -- L_147706495/LConn2
  L_147706495/LConn3 -- T_147706495_220000_/RConn3 -- bus420/LConn1
  T_279711874__/RConn1 -- L_279711874/LConn1
  T_279711874__/RConn2 -- L_279711874/LConn2
  L_279711874/LConn3 -- T_279711874__/RConn3 -- bus421/LConn1
  T_323106340_220000_/RConn1 -- L_323106340/LConn1
  T_323106340_220000_/RConn2 -- L_323106340/LConn2
  L_323106340/LConn3 -- T_323106340_220000_/RConn3 -- bus422/LConn1
  T_277880964__/RConn1 -- L_277880964/LConn1
  T_277880964__/RConn2 -- L_277880964/LConn2
  L_277880964/LConn3 -- T_277880964__/RConn3 -- bus423/LConn1
  T_365843497__/RConn1 -- L_365843497/LConn1
  T_365843497__/RConn2 -- L_365843497/LConn2
  L_365843497/LConn3 -- T_365843497__/RConn3 -- bus424/LConn1
  T_258077674_220000_/RConn1 -- L_258077674/LConn1
  T_258077674_220000_/RConn2 -- L_258077674/LConn2
  L_258077674/LConn3 -- T_258077674_220000_/RConn3 -- bus425/LConn1
  T_279442214__/RConn1 -- L_279442214/LConn1
  T_279442214__/RConn2 -- L_279442214/LConn2
  L_279442214/LConn3 -- T_279442214__/RConn3 -- bus426/LConn1
  T_189145223_220000_/RConn1 -- L_189145223/LConn1
  T_189145223_220000_/RConn2 -- L_189145223/LConn2
  L_189145223/LConn3 -- T_189145223_220000_/RConn3 -- bus427/LConn1
  T_189139925_220000_/RConn1 -- L_189139925/LConn1
  T_189139925_220000_/RConn2 -- L_189139925/LConn2
  L_189139925/LConn3 -- T_189139925_220000_/RConn3 -- bus428/LConn1
  T_315303020_220000_/RConn1 -- L_315303020/LConn1
  T_315303020_220000_/RConn2 -- L_315303020/LConn2
  L_315303020/LConn3 -- T_315303020_220000_/RConn3 -- bus429/LConn1
  T_383977880__/RConn1 -- L_383977880/LConn1
  T_383977880__/RConn2 -- L_383977880/LConn2
  L_383977880/LConn3 -- T_383977880__/RConn3 -- bus430/LConn1
  T_313944391_220000_/RConn1 -- L_313944391/LConn1
  T_313944391_220000_/RConn2 -- L_313944391/LConn2
  L_313944391/LConn3 -- T_313944391_220000_/RConn3 -- bus431/LConn1
  T_336382462__/RConn1 -- L_336382462/LConn1
  T_336382462__/RConn2 -- L_336382462/LConn2
  L_336382462/LConn3 -- T_336382462__/RConn3 -- bus432/LConn1
  T_384012825__/RConn1 -- L_384012825/LConn1
  T_384012825__/RConn2 -- L_384012825/LConn2
  L_384012825/LConn3 -- T_384012825__/RConn3 -- bus433/LConn1
  T_314000703_220000_/RConn1 -- L_314000703/LConn1
  T_314000703_220000_/RConn2 -- L_314000703/LConn2
  L_314000703/LConn3 -- T_314000703_220000_/RConn3 -- bus434/LConn1
  T_160440345__伏陵变电站/RConn1 -- L_160440345/LConn1
  T_160440345__伏陵变电站/RConn2 -- L_160440345/LConn2
  L_160440345/LConn3 -- T_160440345__伏陵变电站/RConn3 -- bus435/LConn1
  T_279946098__/RConn1 -- L_279946098/LConn1
  T_279946098__/RConn2 -- L_279946098/LConn2
  L_279946098/LConn3 -- T_279946098__/RConn3 -- bus436/LConn1
  T_163162788__/RConn1 -- L_163162788/LConn1
  T_163162788__/RConn2 -- L_163162788/LConn2
  L_163162788/LConn3 -- T_163162788__/RConn3 -- bus437/LConn1
  T_163162791__/RConn1 -- L_163162791/LConn1
  T_163162791__/RConn2 -- L_163162791/LConn2
  L_163162791/LConn3 -- T_163162791__/RConn3 -- bus438/LConn1
  T_132503211__/RConn1 -- L_132503211/LConn1
  T_132503211__/RConn2 -- L_132503211/LConn2
  L_132503211/LConn3 -- T_132503211__/RConn3 -- bus439/LConn1
  T_128727215__/RConn1 -- L_128727215/LConn1
  T_128727215__/RConn2 -- L_128727215/LConn2
  L_128727215/LConn3 -- T_128727215__/RConn3 -- bus440/LConn1
  T_132312011__/RConn1 -- L_132312011/LConn1
  T_132312011__/RConn2 -- L_132312011/LConn2
  L_132312011/LConn3 -- T_132312011__/RConn3 -- bus441/LConn1
  T_322733769_220000_/RConn1 -- L_322733769/LConn1
  T_322733769_220000_/RConn2 -- L_322733769/LConn2
  L_322733769/LConn3 -- T_322733769_220000_/RConn3 -- bus442/LConn1
  T_171491187__/RConn1 -- L_171491187/LConn1
  T_171491187__/RConn2 -- L_171491187/LConn2
  L_171491187/LConn3 -- T_171491187__/RConn3 -- bus443/LConn1
  T_131286199_220000_/RConn1 -- L_131286199/LConn1
  T_131286199_220000_/RConn2 -- L_131286199/LConn2
  L_131286199/LConn3 -- T_131286199_220000_/RConn3 -- bus444/LConn1
  T_171514556_220000_/RConn1 -- L_171514556/LConn1
  T_171514556_220000_/RConn2 -- L_171514556/LConn2
  L_171514556/LConn3 -- T_171514556_220000_/RConn3 -- bus445/LConn1
  T_312789337_220000_/RConn1 -- L_312789337/LConn1
  T_312789337_220000_/RConn2 -- L_312789337/LConn2
  L_312789337/LConn3 -- T_312789337_220000_/RConn3 -- bus446/LConn1
  T_170216134__/RConn1 -- L_170216134/LConn1
  T_170216134__/RConn2 -- L_170216134/LConn2
  L_170216134/LConn3 -- T_170216134__/RConn3 -- bus447/LConn1
  T_313944392_220000_/RConn1 -- L_313944392/LConn1
  T_313944392_220000_/RConn2 -- L_313944392/LConn2
  L_313944392/LConn3 -- T_313944392_220000_/RConn3 -- bus448/LConn1
  T_313672407_500000_/RConn1 -- L_313672407/LConn1
  T_313672407_500000_/RConn2 -- L_313672407/LConn2
  L_313672407/LConn3 -- T_313672407_500000_/RConn3 -- bus449/LConn1
  T_166670643__/RConn1 -- L_166670643/LConn1
  T_166670643__/RConn2 -- L_166670643/LConn2
  L_166670643/LConn3 -- T_166670643__/RConn3 -- bus450/LConn1
  T_280819419__/RConn1 -- L_280819419/LConn1
  T_280819419__/RConn2 -- L_280819419/LConn2
  L_280819419/LConn3 -- T_280819419__/RConn3 -- bus451/LConn1
  T_287236840__/RConn1 -- L_287236840/LConn1
  T_287236840__/RConn2 -- L_287236840/LConn2
  L_287236840/LConn3 -- T_287236840__/RConn3 -- bus452/LConn1
  T_104955692_220000_/RConn1 -- L_104955692/LConn1
  T_104955692_220000_/RConn2 -- L_104955692/LConn2
  L_104955692/LConn3 -- T_104955692_220000_/RConn3 -- bus453/LConn1
  T_170703091__/RConn1 -- L_170703091/LConn1
  T_170703091__/RConn2 -- L_170703091/LConn2
  L_170703091/LConn3 -- T_170703091__/RConn3 -- bus454/LConn1
  T_170703094_220000_/RConn1 -- L_170703094/LConn1
  T_170703094_220000_/RConn2 -- L_170703094/LConn2
  L_170703094/LConn3 -- T_170703094_220000_/RConn3 -- bus455/LConn1
  T_283658122__/RConn1 -- L_283658122/LConn1
  T_283658122__/RConn2 -- L_283658122/LConn2
  L_283658122/LConn3 -- T_283658122__/RConn3 -- bus456/LConn1
  T_286930805__/RConn1 -- L_286930805/LConn1
  T_286930805__/RConn2 -- L_286930805/LConn2
  L_286930805/LConn3 -- T_286930805__/RConn3 -- bus457/LConn1
  T_132428536_220000_/RConn1 -- L_132428536/LConn1
  T_132428536_220000_/RConn2 -- L_132428536/LConn2
  L_132428536/LConn3 -- T_132428536_220000_/RConn3 -- bus458/LConn1
  T_132312010_500000_/RConn1 -- L_132312010/LConn1
  T_132312010_500000_/RConn2 -- L_132312010/LConn2
  L_132312010/LConn3 -- T_132312010_500000_/RConn3 -- bus459/LConn1
  T_333873642_220000_/RConn1 -- L_333873642/LConn1
  T_333873642_220000_/RConn2 -- L_333873642/LConn2
  L_333873642/LConn3 -- T_333873642_220000_/RConn3 -- bus460/LConn1
  T_333873652_500000_/RConn1 -- L_333873652/LConn1
  T_333873652_500000_/RConn2 -- L_333873652/LConn2
  L_333873652/LConn3 -- T_333873652_500000_/RConn3 -- bus461/LConn1
  T_95801089__/RConn1 -- L_95801089/LConn1
  T_95801089__/RConn2 -- L_95801089/LConn2
  L_95801089/LConn3 -- T_95801089__/RConn3 -- bus462/LConn1
  T_106027267_220000_/RConn1 -- L_106027267/LConn1
  T_106027267_220000_/RConn2 -- L_106027267/LConn2
  L_106027267/LConn3 -- T_106027267_220000_/RConn3 -- bus463/LConn1
  T_106027361_220000_/RConn1 -- L_106027361/LConn1
  T_106027361_220000_/RConn2 -- L_106027361/LConn2
  L_106027361/LConn3 -- T_106027361_220000_/RConn3 -- bus464/LConn1
  T_321557804_220000_/RConn1 -- L_321557804/LConn1
  T_321557804_220000_/RConn2 -- L_321557804/LConn2
  L_321557804/LConn3 -- T_321557804_220000_/RConn3 -- bus465/LConn1
  T_314893527_220000_/RConn1 -- L_314893527/LConn1
  T_314893527_220000_/RConn2 -- L_314893527/LConn2
  L_314893527/LConn3 -- T_314893527_220000_/RConn3 -- bus466/LConn1
  T_105894253__/RConn1 -- L_105894253/LConn1
  T_105894253__/RConn2 -- L_105894253/LConn2
  L_105894253/LConn3 -- T_105894253__/RConn3 -- bus467/LConn1
  T_312588761_220000_/RConn1 -- L_312588761/LConn1
  T_312588761_220000_/RConn2 -- L_312588761/LConn2
  L_312588761/LConn3 -- T_312588761_220000_/RConn3 -- bus468/LConn1
  T_322733771__/RConn1 -- L_322733771/LConn1
  T_322733771__/RConn2 -- L_322733771/LConn2
  L_322733771/LConn3 -- T_322733771__/RConn3 -- bus469/LConn1
  T_166670641__/RConn1 -- L_166670641/LConn1
  T_166670641__/RConn2 -- L_166670641/LConn2
  L_166670641/LConn3 -- T_166670641__/RConn3 -- bus470/LConn1
  T_329740587_500000_/RConn1 -- L_329740587/LConn1
  T_329740587_500000_/RConn2 -- L_329740587/LConn2
  L_329740587/LConn3 -- T_329740587_500000_/RConn3 -- bus471/LConn1
  T_149239742_220000_/RConn1 -- L_149239742/LConn1
  T_149239742_220000_/RConn2 -- L_149239742/LConn2
  L_149239742/LConn3 -- T_149239742_220000_/RConn3 -- bus472/LConn1
  T_166670638__/RConn1 -- L_166670638/LConn1
  T_166670638__/RConn2 -- L_166670638/LConn2
  L_166670638/LConn3 -- T_166670638__/RConn3 -- bus473/LConn1
  T_166785368__/RConn1 -- L_166785368/LConn1
  T_166785368__/RConn2 -- L_166785368/LConn2
  L_166785368/LConn3 -- T_166785368__/RConn3 -- bus474/LConn1
  T_162167601__/RConn1 -- L_162167601/LConn1
  T_162167601__/RConn2 -- L_162167601/LConn2
  L_162167601/LConn3 -- T_162167601__/RConn3 -- bus475/LConn1
  T_162167607__/RConn1 -- L_162167607/LConn1
  T_162167607__/RConn2 -- L_162167607/LConn2
  L_162167607/LConn3 -- T_162167607__/RConn3 -- bus476/LConn1
  T_166785367__/RConn1 -- L_166785367/LConn1
  T_166785367__/RConn2 -- L_166785367/LConn2
  L_166785367/LConn3 -- T_166785367__/RConn3 -- bus477/LConn1
  T_148003696__/RConn1 -- L_148003696/LConn1
  T_148003696__/RConn2 -- L_148003696/LConn2
  L_148003696/LConn3 -- T_148003696__/RConn3 -- bus478/LConn1
  T_286930814__/RConn1 -- L_286930814/LConn1
  T_286930814__/RConn2 -- L_286930814/LConn2
  L_286930814/LConn3 -- T_286930814__/RConn3 -- bus479/LConn1
  T_132430141__/RConn1 -- L_132430141/LConn1
  T_132430141__/RConn2 -- L_132430141/LConn2
  L_132430141/LConn3 -- T_132430141__/RConn3 -- bus480/LConn1
  T_287217193__/RConn1 -- L_287217193/LConn1
  T_287217193__/RConn2 -- L_287217193/LConn2
  L_287217193/LConn3 -- T_287217193__/RConn3 -- bus481/LConn1
  T_287217195__/RConn1 -- L_287217195/LConn1
  T_287217195__/RConn2 -- L_287217195/LConn2
  L_287217195/LConn3 -- T_287217195__/RConn3 -- bus482/LConn1
  T_107081025_220000_/RConn1 -- L_107081025/LConn1
  T_107081025_220000_/RConn2 -- L_107081025/LConn2
  L_107081025/LConn3 -- T_107081025_220000_/RConn3 -- bus483/LConn1
  T_107025734__/RConn1 -- L_107025734/LConn1
  T_107025734__/RConn2 -- L_107025734/LConn2
  L_107025734/LConn3 -- T_107025734__/RConn3 -- bus484/LConn1
  T_107025738__/RConn1 -- L_107025738/LConn1
  T_107025738__/RConn2 -- L_107025738/LConn2
  L_107025738/LConn3 -- T_107025738__/RConn3 -- bus485/LConn1
  T_148630855__/RConn1 -- L_148630855/LConn1
  T_148630855__/RConn2 -- L_148630855/LConn2
  L_148630855/LConn3 -- T_148630855__/RConn3 -- bus486/LConn1
  T_148630906__/RConn1 -- L_148630906/LConn1
  T_148630906__/RConn2 -- L_148630906/LConn2
  L_148630906/LConn3 -- T_148630906__/RConn3 -- bus487/LConn1
  T_165791616__/RConn1 -- L_165791616/LConn1
  T_165791616__/RConn2 -- L_165791616/LConn2
  L_165791616/LConn3 -- T_165791616__/RConn3 -- bus488/LConn1
  T_313585533_220000_/RConn1 -- L_313585533/LConn1
  T_313585533_220000_/RConn2 -- L_313585533/LConn2
  L_313585533/LConn3 -- T_313585533_220000_/RConn3 -- bus489/LConn1
  T_439464430__/RConn1 -- L_439464430/LConn1
  T_439464430__/RConn2 -- L_439464430/LConn2
  L_439464430/LConn3 -- T_439464430__/RConn3 -- bus490/LConn1
  T_276589719__/RConn1 -- L_276589719/LConn1
  T_276589719__/RConn2 -- L_276589719/LConn2
  L_276589719/LConn3 -- T_276589719__/RConn3 -- bus491/LConn1
  T_107025757_220000_/RConn1 -- L_107025757/LConn1
  T_107025757_220000_/RConn2 -- L_107025757/LConn2
  L_107025757/LConn3 -- T_107025757_220000_/RConn3 -- bus492/LConn1
  T_137158504_220000_/RConn1 -- L_137158504/LConn1
  T_137158504_220000_/RConn2 -- L_137158504/LConn2
  L_137158504/LConn3 -- T_137158504_220000_/RConn3 -- bus493/LConn1
  T_286930806__/RConn1 -- L_286930806/LConn1
  T_286930806__/RConn2 -- L_286930806/LConn2
  L_286930806/LConn3 -- T_286930806__/RConn3 -- bus494/LConn1
  T_286930848__/RConn1 -- L_286930848/LConn1
  T_286930848__/RConn2 -- L_286930848/LConn2
  L_286930848/LConn3 -- T_286930848__/RConn3 -- bus495/LConn1
  T_107081079_220000_/RConn1 -- L_107081079/LConn1
  T_107081079_220000_/RConn2 -- L_107081079/LConn2
  L_107081079/LConn3 -- T_107081079_220000_/RConn3 -- bus496/LConn1
  T_201195907_220000_/RConn1 -- L_201195907/LConn1
  T_201195907_220000_/RConn2 -- L_201195907/LConn2
  L_201195907/LConn3 -- T_201195907_220000_/RConn3 -- bus497/LConn1
  T_284090317__/RConn1 -- L_284090317/LConn1
  T_284090317__/RConn2 -- L_284090317/LConn2
  L_284090317/LConn3 -- T_284090317__/RConn3 -- bus498/LConn1
  T_128731545_220000_/RConn1 -- L_128731545/LConn1
  T_128731545_220000_/RConn2 -- L_128731545/LConn2
  L_128731545/LConn3 -- T_128731545_220000_/RConn3 -- bus499/LConn1
  T_132311997_220000_/RConn1 -- L_132311997/LConn1
  T_132311997_220000_/RConn2 -- L_132311997/LConn2
  L_132311997/LConn3 -- T_132311997_220000_/RConn3 -- bus500/LConn1
  T_286930851__/RConn1 -- L_286930851/LConn1
  T_286930851__/RConn2 -- L_286930851/LConn2
  L_286930851/LConn3 -- T_286930851__/RConn3 -- bus501/LConn1
  T_223960988__/RConn1 -- L_223960988/LConn1
  T_223960988__/RConn2 -- L_223960988/LConn2
  L_223960988/LConn3 -- T_223960988__/RConn3 -- bus502/LConn1
  T_337055172_500000_/RConn1 -- L_337055172/LConn1
  T_337055172_500000_/RConn2 -- L_337055172/LConn2
  L_337055172/LConn3 -- T_337055172_500000_/RConn3 -- bus503/LConn1
  T_314318262_220000_/RConn1 -- L_314318262/LConn1
  T_314318262_220000_/RConn2 -- L_314318262/LConn2
  L_314318262/LConn3 -- T_314318262_220000_/RConn3 -- bus504/LConn1
  T_284090323__/RConn1 -- L_284090323/LConn1
  T_284090323__/RConn2 -- L_284090323/LConn2
  L_284090323/LConn3 -- T_284090323__/RConn3 -- bus505/LConn1
  T_287200264__/RConn1 -- L_287200264/LConn1
  T_287200264__/RConn2 -- L_287200264/LConn2
  L_287200264/LConn3 -- T_287200264__/RConn3 -- bus506/LConn1
  T_287132220__/RConn1 -- L_287132220/LConn1
  T_287132220__/RConn2 -- L_287132220/LConn2
  L_287132220/LConn3 -- T_287132220__/RConn3 -- bus507/LConn1
  T_194636809__/RConn1 -- L_194636809/LConn1
  T_194636809__/RConn2 -- L_194636809/LConn2
  L_194636809/LConn3 -- T_194636809__/RConn3 -- bus508/LConn1
  T_192701020_500000_/RConn1 -- L_192701020/LConn1
  T_192701020_500000_/RConn2 -- L_192701020/LConn2
  L_192701020/LConn3 -- T_192701020_500000_/RConn3 -- bus509/LConn1
  T_349963792__/RConn1 -- L_349963792/LConn1
  T_349963792__/RConn2 -- L_349963792/LConn2
  L_349963792/LConn3 -- T_349963792__/RConn3 -- bus510/LConn1
  T_143214751__/RConn1 -- L_143214751/LConn1
  T_143214751__/RConn2 -- L_143214751/LConn2
  L_143214751/LConn3 -- T_143214751__/RConn3 -- bus511/LConn1
  T_281631619__/RConn1 -- L_281631619/LConn1
  T_281631619__/RConn2 -- L_281631619/LConn2
  L_281631619/LConn3 -- T_281631619__/RConn3 -- bus512/LConn1
  T_281631607__/RConn1 -- L_281631607/LConn1
  T_281631607__/RConn2 -- L_281631607/LConn2
  L_281631607/LConn3 -- T_281631607__/RConn3 -- bus513/LConn1
  T_161803803_500000_/RConn1 -- L_161803803/LConn1
  T_161803803_500000_/RConn2 -- L_161803803/LConn2
  L_161803803/LConn3 -- T_161803803_500000_/RConn3 -- bus514/LConn1
  T_328430431_500000_/RConn1 -- L_328430431/LConn1
  T_328430431_500000_/RConn2 -- L_328430431/LConn2
  L_328430431/LConn3 -- T_328430431_500000_/RConn3 -- bus515/LConn1
  T_212792929__/RConn1 -- L_212792929/LConn1
  T_212792929__/RConn2 -- L_212792929/LConn2
  L_212792929/LConn3 -- T_212792929__/RConn3 -- bus516/LConn1
  T_317023804_500000_/RConn1 -- L_317023804/LConn1
  T_317023804_500000_/RConn2 -- L_317023804/LConn2
  L_317023804/LConn3 -- T_317023804_500000_/RConn3 -- bus517/LConn1
  T_251393861_500000_/RConn1 -- L_251393861/LConn1
  T_251393861_500000_/RConn2 -- L_251393861/LConn2
  L_251393861/LConn3 -- T_251393861_500000_/RConn3 -- bus518/LConn1
  T_313528393_500000_/RConn1 -- L_313528393/LConn1
  T_313528393_500000_/RConn2 -- L_313528393/LConn2
  L_313528393/LConn3 -- T_313528393_500000_/RConn3 -- bus519/LConn1
  T_313528394_500000_/RConn1 -- L_313528394/LConn1
  T_313528394_500000_/RConn2 -- L_313528394/LConn2
  L_313528394/LConn3 -- T_313528394_500000_/RConn3 -- bus520/LConn1
  T_304003393_500000_/RConn1 -- L_304003393/LConn1
  T_304003393_500000_/RConn2 -- L_304003393/LConn2
  L_304003393/LConn3 -- T_304003393_500000_/RConn3 -- bus521/LConn1
  T_319236194_500000_/RConn1 -- L_319236194/LConn1
  T_319236194_500000_/RConn2 -- L_319236194/LConn2
  L_319236194/LConn3 -- T_319236194_500000_/RConn3 -- bus522/LConn1
  T_321597229_500000_/RConn1 -- L_321597229/LConn1
  T_321597229_500000_/RConn2 -- L_321597229/LConn2
  L_321597229/LConn3 -- T_321597229_500000_/RConn3 -- bus523/LConn1
  T_264811102_500000_/RConn1 -- L_264811102/LConn1
  T_264811102_500000_/RConn2 -- L_264811102/LConn2
  L_264811102/LConn3 -- T_264811102_500000_/RConn3 -- bus524/LConn1
  T_302492014__/RConn1 -- L_302492014/LConn1
  T_302492014__/RConn2 -- L_302492014/LConn2
  L_302492014/LConn3 -- T_302492014__/RConn3 -- bus525/LConn1
  T_171491177_500000_漕泾/RConn1 -- L_171491177/LConn1
  T_171491177_500000_漕泾/RConn2 -- L_171491177/LConn2
  L_171491177/LConn3 -- T_171491177_500000_漕泾/RConn3 -- bus526/LConn1
  T_424682264__/RConn1 -- L_424682264/LConn1
  T_424682264__/RConn2 -- L_424682264/LConn2
  L_424682264/LConn3 -- T_424682264__/RConn3 -- bus527/LConn1
  T_171491189__/RConn1 -- L_171491189/LConn1
  T_171491189__/RConn2 -- L_171491189/LConn2
  L_171491189/LConn3 -- T_171491189__/RConn3 -- bus528/LConn1
  T_313316283_500000_/RConn1 -- L_313316283/LConn1
  T_313316283_500000_/RConn2 -- L_313316283/LConn2
  L_313316283/LConn3 -- T_313316283_500000_/RConn3 -- bus529/LConn1
  T_148104555__/RConn1 -- L_148104555/LConn1
  T_148104555__/RConn2 -- L_148104555/LConn2
  L_148104555/LConn3 -- T_148104555__/RConn3 -- bus530/LConn1
  T_325720933_500000_/RConn1 -- L_325720933/LConn1
  T_325720933_500000_/RConn2 -- L_325720933/LConn2
  L_325720933/LConn3 -- T_325720933_500000_/RConn3 -- bus531/LConn1
  T_314866321_500000_/RConn1 -- L_314866321/LConn1
  T_314866321_500000_/RConn2 -- L_314866321/LConn2
  L_314866321/LConn3 -- T_314866321_500000_/RConn3 -- bus532/LConn1
  T_317280360__/RConn1 -- L_317280360/LConn1
  T_317280360__/RConn2 -- L_317280360/LConn2
  L_317280360/LConn3 -- T_317280360__/RConn3 -- bus533/LConn1
  T_327333768_500000_/RConn1 -- L_327333768/LConn1
  T_327333768_500000_/RConn2 -- L_327333768/LConn2
  L_327333768/LConn3 -- T_327333768_500000_/RConn3 -- bus534/LConn1
  T_261427501__/RConn1 -- L_261427501/LConn1
  T_261427501__/RConn2 -- L_261427501/LConn2
  L_261427501/LConn3 -- T_261427501__/RConn3 -- bus535/LConn1
  T_278062437__/RConn1 -- L_278062437/LConn1
  T_278062437__/RConn2 -- L_278062437/LConn2
  L_278062437/LConn3 -- T_278062437__/RConn3 -- bus536/LConn1
  T_312852542_500000_/RConn1 -- L_312852542/LConn1
  T_312852542_500000_/RConn2 -- L_312852542/LConn2
  L_312852542/LConn3 -- T_312852542_500000_/RConn3 -- bus537/LConn1
  T_325720937_500000_/RConn1 -- L_325720937/LConn1
  T_325720937_500000_/RConn2 -- L_325720937/LConn2
  L_325720937/LConn3 -- T_325720937_500000_/RConn3 -- bus538/LConn1
  T_146077915__/RConn1 -- L_146077915/LConn1
  T_146077915__/RConn2 -- L_146077915/LConn2
  L_146077915/LConn3 -- T_146077915__/RConn3 -- bus539/LConn1
  T_312922833_500000_/RConn1 -- L_312922833/LConn1
  T_312922833_500000_/RConn2 -- L_312922833/LConn2
  L_312922833/LConn3 -- T_312922833_500000_/RConn3 -- bus540/LConn1
  T_132424995__/RConn1 -- L_132424995/LConn1
  T_132424995__/RConn2 -- L_132424995/LConn2
  L_132424995/LConn3 -- T_132424995__/RConn3 -- bus541/LConn1
  T_323032993_500000_/RConn1 -- L_323032993/LConn1
  T_323032993_500000_/RConn2 -- L_323032993/LConn2
  L_323032993/LConn3 -- T_323032993_500000_/RConn3 -- bus542/LConn1
  T_322892827_500000_/RConn1 -- L_322892827/LConn1
  T_322892827_500000_/RConn2 -- L_322892827/LConn2
  L_322892827/LConn3 -- T_322892827_500000_/RConn3 -- bus543/LConn1
  T_323016571_500000_/RConn1 -- L_323016571/LConn1
  T_323016571_500000_/RConn2 -- L_323016571/LConn2
  L_323016571/LConn3 -- T_323016571_500000_/RConn3 -- bus544/LConn1
  T_279809227__/RConn1 -- L_279809227/LConn1
  T_279809227__/RConn2 -- L_279809227/LConn2
  L_279809227/LConn3 -- T_279809227__/RConn3 -- bus545/LConn1
  T_232408714_500000_里木栅500KV超高压变电站/RConn1 -- L_232408714/LConn1
  T_232408714_500000_里木栅500KV超高压变电站/RConn2 -- L_232408714/LConn2
  L_232408714/LConn3 -- T_232408714_500000_里木栅500KV超高压变电站/RConn3 -- bus546/LConn1
  T_323698983_500000_/RConn1 -- L_323698983/LConn1
  T_323698983_500000_/RConn2 -- L_323698983/LConn2
  L_323698983/LConn3 -- T_323698983_500000_/RConn3 -- bus547/LConn1
  T_323965697_500000_/RConn1 -- L_323965697/LConn1
  T_323965697_500000_/RConn2 -- L_323965697/LConn2
  L_323965697/LConn3 -- T_323965697_500000_/RConn3 -- bus548/LConn1
  T_323880677_500000_/RConn1 -- L_323880677/LConn1
  T_323880677_500000_/RConn2 -- L_323880677/LConn2
  L_323880677/LConn3 -- T_323880677_500000_/RConn3 -- bus549/LConn1
  T_287076644__/RConn1 -- L_287076644/LConn1
  T_287076644__/RConn2 -- L_287076644/LConn2
  L_287076644/LConn3 -- T_287076644__/RConn3 -- bus550/LConn1
  T_287076645__/RConn1 -- L_287076645/LConn1
  T_287076645__/RConn2 -- L_287076645/LConn2
  L_287076645/LConn3 -- T_287076645__/RConn3 -- bus551/LConn1
  T_314351248_500000_/RConn1 -- L_314351248/LConn1
  T_314351248_500000_/RConn2 -- L_314351248/LConn2
  L_314351248/LConn3 -- T_314351248_500000_/RConn3 -- bus552/LConn1
  T_313954993_500000_/RConn1 -- L_313954993/LConn1
  T_313954993_500000_/RConn2 -- L_313954993/LConn2
  L_313954993/LConn3 -- T_313954993_500000_/RConn3 -- bus553/LConn1
  T_157709467__/RConn1 -- L_157709467/LConn1
  T_157709467__/RConn2 -- L_157709467/LConn2
  L_157709467/LConn3 -- T_157709467__/RConn3 -- bus554/LConn1
  T_276719460__/RConn1 -- L_276719460/LConn1
  T_276719460__/RConn2 -- L_276719460/LConn2
  L_276719460/LConn3 -- T_276719460__/RConn3 -- bus555/LConn1
  T_128727214__/RConn1 -- L_128727214/LConn1
  T_128727214__/RConn2 -- L_128727214/LConn2
  L_128727214/LConn3 -- T_128727214__/RConn3 -- bus556/LConn1
  T_171491186__/RConn1 -- L_171491186/LConn1
  T_171491186__/RConn2 -- L_171491186/LConn2
  L_171491186/LConn3 -- T_171491186__/RConn3 -- bus557/LConn1
  T_312583866_500000_/RConn1 -- L_312583866/LConn1
  T_312583866_500000_/RConn2 -- L_312583866/LConn2
  L_312583866/LConn3 -- T_312583866_500000_/RConn3 -- bus558/LConn1
  T_315071478_500000_/RConn1 -- L_315071478/LConn1
  T_315071478_500000_/RConn2 -- L_315071478/LConn2
  L_315071478/LConn3 -- T_315071478_500000_/RConn3 -- bus559/LConn1
  T_254904701_500000_/RConn1 -- L_254904701/LConn1
  T_254904701_500000_/RConn2 -- L_254904701/LConn2
  L_254904701/LConn3 -- T_254904701_500000_/RConn3 -- bus560/LConn1
  T_79198909_500000_/RConn1 -- L_79198909/LConn1
  T_79198909_500000_/RConn2 -- L_79198909/LConn2
  L_79198909/LConn3 -- T_79198909_500000_/RConn3 -- bus561/LConn1
  T_312922832_500000_/RConn1 -- L_312922832/LConn1
  T_312922832_500000_/RConn2 -- L_312922832/LConn2
  L_312922832/LConn3 -- T_312922832_500000_/RConn3 -- bus562/LConn1
  T_163357534__/RConn1 -- L_163357534/LConn1
  T_163357534__/RConn2 -- L_163357534/LConn2
  L_163357534/LConn3 -- T_163357534__/RConn3 -- bus563/LConn1
  T_334707427__/RConn1 -- L_334707427/LConn1
  T_334707427__/RConn2 -- L_334707427/LConn2
  L_334707427/LConn3 -- T_334707427__/RConn3 -- bus564/LConn1
  T_286137154__/RConn1 -- L_286137154/LConn1
  T_286137154__/RConn2 -- L_286137154/LConn2
  L_286137154/LConn3 -- T_286137154__/RConn3 -- bus565/LConn1
  T_303677167__/RConn1 -- L_303677167/LConn1
  T_303677167__/RConn2 -- L_303677167/LConn2
  L_303677167/LConn3 -- T_303677167__/RConn3 -- bus566/LConn1
  T_283658133__/RConn1 -- L_283658133/LConn1
  T_283658133__/RConn2 -- L_283658133/LConn2
  L_283658133/LConn3 -- T_283658133__/RConn3 -- bus567/LConn1
  T_300336767__/RConn1 -- L_300336767/LConn1
  T_300336767__/RConn2 -- L_300336767/LConn2
  L_300336767/LConn3 -- T_300336767__/RConn3 -- bus568/LConn1
  T_301061895__/RConn1 -- L_301061895/LConn1
  T_301061895__/RConn2 -- L_301061895/LConn2
  L_301061895/LConn3 -- T_301061895__/RConn3 -- bus569/LConn1
  T_327908612_500000_/RConn1 -- L_327908612/LConn1
  T_327908612_500000_/RConn2 -- L_327908612/LConn2
  L_327908612/LConn3 -- T_327908612_500000_/RConn3 -- bus570/LConn1
  T_424682265__/RConn1 -- L_424682265/LConn1
  T_424682265__/RConn2 -- L_424682265/LConn2
  L_424682265/LConn3 -- T_424682265__/RConn3 -- bus571/LConn1
  T_323032986__/RConn1 -- L_323032986/LConn1
  T_323032986__/RConn2 -- L_323032986/LConn2
  L_323032986/LConn3 -- T_323032986__/RConn3 -- bus572/LConn1
  T_424682272__/RConn1 -- L_424682272/LConn1
  T_424682272__/RConn2 -- L_424682272/LConn2
  L_424682272/LConn3 -- T_424682272__/RConn3 -- bus573/LConn1
  T_315071484_500000_/RConn1 -- L_315071484/LConn1
  T_315071484_500000_/RConn2 -- L_315071484/LConn2
  L_315071484/LConn3 -- T_315071484_500000_/RConn3 -- bus574/LConn1
  T_321690480_500000_/RConn1 -- L_321690480/LConn1
  T_321690480_500000_/RConn2 -- L_321690480/LConn2
  L_321690480/LConn3 -- T_321690480_500000_/RConn3 -- bus575/LConn1
  T_132503439_220000_/RConn1 -- L_132503439/LConn1
  T_132503439_220000_/RConn2 -- L_132503439/LConn2
  L_132503439/LConn3 -- T_132503439_220000_/RConn3 -- bus576/LConn1
  T_163357508__Zhengping_Static_Inverter_Plant/RConn1 -- L_163357508/LConn1
  T_163357508__Zhengping_Static_Inverter_Plant/RConn2 -- L_163357508/LConn2
  L_163357508/LConn3 -- T_163357508__Zhengping_Static_Inverter_Plant/RConn3 -- bus577/LConn1
  T_314164572_500000_/RConn1 -- L_314164572/LConn1
  T_314164572_500000_/RConn2 -- L_314164572/LConn2
  L_314164572/LConn3 -- T_314164572_500000_/RConn3 -- bus578/LConn1
  T_321690463_500000_/RConn1 -- L_321690463/LConn1
  T_321690463_500000_/RConn2 -- L_321690463/LConn2
  L_321690463/LConn3 -- T_321690463_500000_/RConn3 -- bus579/LConn1
  T_181090227_500000;220000_/RConn1 -- L_181090227/LConn1
  T_181090227_500000;220000_/RConn2 -- L_181090227/LConn2
  L_181090227/LConn3 -- T_181090227_500000;220000_/RConn3 -- bus580/LConn1
  T_312925118_500000_/RConn1 -- L_312925118/LConn1
  T_312925118_500000_/RConn2 -- L_312925118/LConn2
  L_312925118/LConn3 -- T_312925118_500000_/RConn3 -- bus581/LConn1
  T_314606532_500000_/RConn1 -- L_314606532/LConn1
  T_314606532_500000_/RConn2 -- L_314606532/LConn2
  L_314606532/LConn3 -- T_314606532_500000_/RConn3 -- bus582/LConn1
  T_287200191__/RConn1 -- L_287200191/LConn1
  T_287200191__/RConn2 -- L_287200191/LConn2
  L_287200191/LConn3 -- T_287200191__/RConn3 -- bus583/LConn1
